simulink library "ammclib_bam_S32K3xx"  (R2016a)
(part 23 of 50)

      |     delete_block([gcb, '/fltInK_1_D']);
      |     add_block('built-in/Inport', [gcb, '/fltInK_1_D'], 'Position', pos, 'Orientation', orient, 'OutDataTypeStr', 'single');
      | 
      |     pos = get_param([gcb, '/fltPropGain_Q'], 'Position');
      |     orient = get_param([gcb, '/fltPropGain_Q'], 'Orientation');
      |     delete_block([gcb, '/fltPropGain_Q']);
      |     add_block('built-in/Inport', [gcb, '/fltPropGain_Q'], 'Position', pos, 'Orientation', orient, 'OutDataTypeStr', 'single');
      | 
      |     pos = get_param([gcb, '/fltIntegGain_Q'], 'Position');
      |     orient = get_param([gcb, '/fltIntegGain_Q'], 'Orientation');
      |     delete_block([gcb, '/fltIntegGain_Q']);
      |     add_block('built-in/Inport', [gcb, '/fltIntegGain_Q'], 'Position', pos, 'Orientation', orient, 'OutDataTypeStr', 'single');
      | 
      |     pos = get_param([gcb, '/fltIntegPartK_1_Q'], 'Position');
      |     orient = get_param([gcb, '/fltIntegPartK_1_Q'], 'Orientation');
      |     delete_block([gcb, '/fltIntegPartK_1_Q']);
      |     add_block('built-in/Inport', [gcb, '/fltIntegPartK_1_Q'], 'Position', pos, 'Orientation', orient, 'OutDataTypeStr', 'single');
      | 
      |     pos = get_param([gcb, '/fltInK_1_Q'], 'Position');
      |     orient = get_param([gcb, '/fltInK_1_Q'], 'Orientation');
      |     delete_block([gcb, '/fltInK_1_Q']);
      |     add_block('built-in/Inport', [gcb, '/fltInK_1_Q'], 'Position', pos, 'Orientation', orient, 'OutDataTypeStr', 'single');
      | 
      | 
      | 
      |     pos = get_param([gcb '/fltIntegPartK_1_D_Out'], 'Position');
      |     orient = get_param([gcb '/fltIntegPartK_1_D_Out'], 'Orientation');
      |     delete_block([gcb '/fltIntegPartK_1_D_Out']);
      |     add_block('built-in/Outport', [gcb '/fltIntegPartK_1_D_Out'], 'Position', pos, 'Orientation', orient);
      | 
      |     pos = get_param([gcb '/fltInK_1_D_Out'], 'Position');
      |     orient = get_param([gcb '/fltInK_1_D_Out'], 'Orientation');
      |     delete_block([gcb '/fltInK_1_D_Out']);
      |     add_block('built-in/Outport', [gcb '/fltInK_1_D_Out'], 'Position', pos, 'Orientation', orient);
      | 
      |     pos = get_param([gcb '/fltIntegPartK_1_Q_Out'], 'Position');
      |     orient = get_param([gcb '/fltIntegPartK_1_Q_Out'], 'Orientation');
      |     delete_block([gcb '/fltIntegPartK_1_Q_Out']);
      |     add_block('built-in/Outport', [gcb '/fltIntegPartK_1_Q_Out'], 'Position', pos, 'Orientation', orient);
      | 
      |     pos = get_param([gcb '/fltInK_1_Q_Out'], 'Position');
      |     orient = get_param([gcb '/fltInK_1_Q_Out'], 'Orientation');
      |     delete_block([gcb '/fltInK_1_Q_Out']);
      |     add_block('built-in/Outport', [gcb '/fltInK_1_Q_Out'], 'Position', pos, 'Orientation', orient);
      | 
      | 
      |     pmask=Simulink.Mask.get(gcb);
      |     pctrl=pmask.getParameter('SampleTime');
      |     pctrl.set('TypeOptions',{'fltUDcBus/SampleTime','pIDQReq/SampleTime','pIDQFbck/SampleTime','fltControllerPIpAWDOut_preset/SampleTime','fltControllerPIpAWQOut_preset/SampleTime','fltPropGain_D/SampleTime','fltIntegGain_D/SampleTime','fltIntegPartK_1_D/SampleTime','fltInK_1_D/SampleTime','fltPropGain_Q/SampleTime','fltIntegGain_Q/SampleTime','fltIntegPartK_1_Q/SampleTime','fltInK_1_Q/SampleTime'});
      | 
      |     set_param([gcb '/fltUDcBus'], 'Port', '1');
      |     set_param([gcb '/pIDQReq'], 'Port', '2');
      |     set_param([gcb '/pIDQFbck'], 'Port', '3');
      |     set_param([gcb '/fltControllerPIpAWDOut_preset'], 'Port', '4');
      |     set_param([gcb '/fltControllerPIpAWQOut_preset'], 'Port', '5');
      |     set_param([gcb '/fltPropGain_D'], 'Port', '6');
      |     set_param([gcb '/fltIntegGain_D'], 'Port', '7');
      |     set_param([gcb '/fltIntegPartK_1_D'], 'Port', '8');
      |     set_param([gcb '/fltInK_1_D'], 'Port', '9');
      |     set_param([gcb '/fltPropGain_Q'], 'Port', '10');
      |     set_param([gcb '/fltIntegGain_Q'], 'Port', '11');
      |     set_param([gcb '/fltIntegPartK_1_Q'], 'Port', '12');
      |     set_param([gcb '/fltInK_1_Q'], 'Port', '13');
      | 
      |     tmpOutCnt=0;
      |     tmpOutCnt=tmpOutCnt+1;
      |     set_param([gcb '/pUDQReq'], 'Port', num2str(tmpOutCnt));
      |     tmpOutCnt=tmpOutCnt+1;
      |     set_param([gcb '/fltUQLim'], 'Port', num2str(tmpOutCnt));
      |     tmpOutCnt=tmpOutCnt+1;
      |     set_param([gcb '/fltIntegPartK_1_D_Out'], 'Port', num2str(tmpOutCnt));
      |     tmpOutCnt=tmpOutCnt+1;
      |     set_param([gcb '/fltInK_1_D_Out'], 'Port', num2str(tmpOutCnt));
      |     tmpOutCnt=tmpOutCnt+1;
      |     set_param([gcb '/fltIntegPartK_1_Q_Out'], 'Port', num2str(tmpOutCnt));
      |     tmpOutCnt=tmpOutCnt+1;
      |     set_param([gcb '/fltInK_1_Q_Out'], 'Port', num2str(tmpOutCnt));
      | 
      |     set_param(gcb,'MaskEnables',{'on','on','on','off','off','off','off','off','off','off','off','off','off','off'});
      | 
      |     if (posblk(4) - posblk(2)) < 350
      |       height = 350;
      |       set_param(gcb,'Position',[posblk(1), posblk(2), posblk(3), posblk(2)+height])
      |     end
      |   end
      | end
      settings: RTWSystemCode=Inline
      mask Help: web([fileparts(which('ammclib_bam_S32K3xx.slx')) '/../doc/S32K3XXMCLUG.pdf'], '-browser')
      mask TypeOptions showStates: Hide (faster execution) | Show (allows debugging; connect feedback loops manually)
      mask Callback showStates:
      | maskStr=get_param(gcb,'showStates');
      | if strcmp(maskStr,'Hide (faster execution)')
      |   if strcmp(get_param([gcb '/fltPropGain_D'], 'BlockType'), 'Inport')
      |     autoCalcEn=get_param(gcb,'autoCalcEn');
      |     if strcmp(autoCalcEn,'on')
      |       set_param(gcb,'MaskEnables',{'on','on','on','on','on','on','on','on','on','on','on','on','on','off'});
      |     else
      |       set_param(gcb,'MaskEnables',{'on','on','on','off','off','off','off','off','on','on','on','on','on','off'});
      |     end
      |   end
      | else
      |   if strcmp(get_param([gcb '/fltPropGain_D'], 'BlockType'), 'Ground')
      |     set_param(gcb,'MaskEnables',{'on','on','on','off','off','off','off','off','off','off','off','off','off','off'});
      |   end
      | end
      mask TypeOptions resetStatesEnable: Pre-set according to the first set of inputs after reset | Clear to zero
      mask TypeOptions SampleTime: fltUDcBus/SampleTime | pIDQReq/SampleTime | pIDQFbck/SampleTime | fltControllerPIpAWDOut_preset/SampleTime | fltControllerPIpAWQOut_preset/SampleTime
      mask Callback SampleTime:
      | p=Simulink.Mask.get(gcb);
      | hintText=p.getDialogControl('timeHint');
      | SampleTime=Simulink.data.evalinGlobal(bdroot,get_param(gcb,'SampleTime'));
      | SampleTime_1=str2double(get_param(gcb,'SampleTime_1'));
      | if (((SampleTime==-1) && (~contains(hintText.Prompt,'inherited'))) || ...
      |     ((SampleTime~=-1) && contains(hintText.Prompt,'inherited')) || ...
      |     ((SampleTime~=-1) && (SampleTime_1~=SampleTime)) || ...
      |     ((SampleTime_1~=-1) && contains(hintText.Prompt,'yet')))
      |   if ((SampleTime==-1) && (~contains(hintText.Prompt,'inherited')))
      |     set_param(gcb,'SampleTime_1',num2str(NaN));
      |     SampleTime_1=NaN;
      |   end
      |   if (SampleTime~=-1)
      |     set_param(gcb,'SampleTime_1',num2str(SampleTime));
      |     SampleTime_1=SampleTime;
      |   end
      |   autoCalcEn=get_param(gcb,'autoCalcEn');
      |   if strcmp(autoCalcEn,'on')
      |     p=Simulink.Mask.get(gcb);
      |     hintText=p.getDialogControl('timeHint');
      |     if SampleTime==-1
      |       SampleTime=SampleTime_1;
      |       if isnan(SampleTime)
      |         hintText.Prompt='Note: Implementation parameters cannot be calculated yet because the block''s inherited sample time is unknown. Simulink will update the sample time when you run the simulation.';
      |       else
      |         hintText.Prompt='Caution: Implementation parameters depend on inherited sample time. Make sure that the sample time of the block''s inputs corresponds to the sampling period in the target application.';
      |       end
      |     else
      |       hintText.Prompt='Caution: Implementation parameters depend on the sample time. Make sure that the simulation time step corresponds to the sampling period in the target application.';
      |     end
      |     fltPropGain_D_bkup=get_param(gcb,'fltPropGain_D');
      |     fltIntegGain_D_bkup=get_param(gcb,'fltIntegGain_D');
      |     fltPropGain_Q_bkup=get_param(gcb,'fltPropGain_Q');
      |     fltIntegGain_Q_bkup=get_param(gcb,'fltIntegGain_Q');
      |     if0=Simulink.data.evalinGlobal(bdroot,get_param(gcb,'if0'));
      |     iksi=Simulink.data.evalinGlobal(bdroot,get_param(gcb,'iksi'));
      |     Ld=Simulink.data.evalinGlobal(bdroot,get_param(gcb,'Ld'));
      |     Lq=Simulink.data.evalinGlobal(bdroot,get_param(gcb,'Lq'));
      |     Rs=Simulink.data.evalinGlobal(bdroot,get_param(gcb,'Rs'));
      |     if (if0<=0)
      |       warning('Natural frequency f0 must be positive.');
      |     end
      |     if (iksi<=0)
      |       warning('Current loop attenuation must be positive.');
      |     end
      |     if (iksi>1)
      |       warning('Current loop attenuation must not exceed 1.');
      |     end
      |     if (Ld<=0)
      |       warning('Inductance Ld must be positive.');
      |     end
      |     if (Lq<=0)
      |       warning('Inductance Lq must be positive.');
      |     end
      |     if (Rs<0)
      |       warning('Resistance Rs must be non-negative.');
      |     end
      |     w0=6.283185307179586*if0;
      |     pgainD=2.0*iksi*w0*Ld-Rs;
      |     igainD=w0*w0*Ld;
      |     pgainQ=2.0*iksi*w0*Lq-Rs;
      |     igainQ=w0*w0*Lq;
      |     fltPropGain_D=pgainD;
      |     fltIntegGain_D=igainD*SampleTime*0.5;
      |     fltPropGain_Q=pgainQ;
      |     fltIntegGain_Q=igainQ*SampleTime*0.5;
      |     if isnan(fltPropGain_D)
      |       if ~strcmp(fltPropGain_D_bkup,'0')
      |         set_param(gcb,'fltPropGain_D','0');
      |       end
      |     else
      |       tmps=num2str(fltPropGain_D);
      |       if ~strcmp(fltPropGain_D_bkup,tmps)
      |         set_param(gcb,'fltPropGain_D',tmps);
      |       end
      |     end
      |     if isnan(fltIntegGain_D)
      |       if ~strcmp(fltIntegGain_D_bkup,'0')
      |         set_param(gcb,'fltIntegGain_D','0');
      |       end
      |     else
      |       tmps=num2str(fltIntegGain_D);
      |       if ~strcmp(fltIntegGain_D_bkup,tmps)
      |         set_param(gcb,'fltIntegGain_D',tmps);
      |       end
      |     end
      |     if isnan(fltPropGain_Q)
      |       if ~strcmp(fltPropGain_Q_bkup,'0')
      |         set_param(gcb,'fltPropGain_Q','0');
      |       end
      |     else
      |       tmps=num2str(fltPropGain_Q);
      |       if ~strcmp(fltPropGain_Q_bkup,tmps)
      |         set_param(gcb,'fltPropGain_Q',tmps);
      |       end
      |     end
      |     if isnan(fltIntegGain_Q)
      |       if ~strcmp(fltIntegGain_Q_bkup,'0')
      |         set_param(gcb,'fltIntegGain_Q','0');
      |       end
      |     else
      |       tmps=num2str(fltIntegGain_Q);
      |       if ~strcmp(fltIntegGain_Q_bkup,tmps)
      |         set_param(gcb,'fltIntegGain_Q',tmps);
      |       end
      |     end
      |   end
      | end
      mask Callback if0:
      | autoCalcEn=get_param(gcb,'autoCalcEn');
      | if strcmp(autoCalcEn,'on')
      |   SampleTime=Simulink.data.evalinGlobal(bdroot,get_param(gcb,'SampleTime'));
      |   if (SampleTime==-1)
      |     SampleTime=str2double(get_param(gcb,'SampleTime_1'));
      |   end
      |   fltPropGain_D_bkup=get_param(gcb,'fltPropGain_D');
      |   fltIntegGain_D_bkup=get_param(gcb,'fltIntegGain_D');
      |   fltPropGain_Q_bkup=get_param(gcb,'fltPropGain_Q');
      |   fltIntegGain_Q_bkup=get_param(gcb,'fltIntegGain_Q');
      |   if0=Simulink.data.evalinGlobal(bdroot,get_param(gcb,'if0'));
      |   iksi=Simulink.data.evalinGlobal(bdroot,get_param(gcb,'iksi'));
      |   Ld=Simulink.data.evalinGlobal(bdroot,get_param(gcb,'Ld'));
      |   Lq=Simulink.data.evalinGlobal(bdroot,get_param(gcb,'Lq'));
      |   Rs=Simulink.data.evalinGlobal(bdroot,get_param(gcb,'Rs'));
      |   if (if0<=0)
      |     warning('Natural frequency f0 must be positive.');
      |   end
      |   if (iksi<=0)
      |     warning('Current loop attenuation must be positive.');
      |   end
      |   if (iksi>1)
      |     warning('Current loop attenuation must not exceed 1.');
      |   end
      |   if (Ld<=0)
      |     warning('Inductance Ld must be positive.');
      |   end
      |   if (Lq<=0)
      |     warning('Inductance Lq must be positive.');
      |   end
      |   if (Rs<0)
      |     warning('Resistance Rs must be non-negative.');
      |   end
      |   w0=6.283185307179586*if0;
      |   pgainD=2.0*iksi*w0*Ld-Rs;
      |   igainD=w0*w0*Ld;
      |   pgainQ=2.0*iksi*w0*Lq-Rs;
      |   igainQ=w0*w0*Lq;
      |   fltPropGain_D=pgainD;
      |   fltIntegGain_D=igainD*SampleTime*0.5;
      |   fltPropGain_Q=pgainQ;
      |   fltIntegGain_Q=igainQ*SampleTime*0.5;
      |   if isnan(fltPropGain_D)
      |     if ~strcmp(fltPropGain_D_bkup,'0')
      |       set_param(gcb,'fltPropGain_D','0');
      |     end
      |   else
      |     tmps=num2str(fltPropGain_D);
      |     if ~strcmp(fltPropGain_D_bkup,tmps)
      |       set_param(gcb,'fltPropGain_D',tmps);
      |     end
      |   end
      |   if isnan(fltIntegGain_D)
      |     if ~strcmp(fltIntegGain_D_bkup,'0')
      |       set_param(gcb,'fltIntegGain_D','0');
      |     end
      |   else
      |     tmps=num2str(fltIntegGain_D);
      |     if ~strcmp(fltIntegGain_D_bkup,tmps)
      |       set_param(gcb,'fltIntegGain_D',tmps);
      |     end
      |   end
      |   if isnan(fltPropGain_Q)
      |     if ~strcmp(fltPropGain_Q_bkup,'0')
      |       set_param(gcb,'fltPropGain_Q','0');
      |     end
      |   else
      |     tmps=num2str(fltPropGain_Q);
      |     if ~strcmp(fltPropGain_Q_bkup,tmps)
      |       set_param(gcb,'fltPropGain_Q',tmps);
      |     end
      |   end
      |   if isnan(fltIntegGain_Q)
      |     if ~strcmp(fltIntegGain_Q_bkup,'0')
      |       set_param(gcb,'fltIntegGain_Q','0');
      |     end
      |   else
      |     tmps=num2str(fltIntegGain_Q);
      |     if ~strcmp(fltIntegGain_Q_bkup,tmps)
      |       set_param(gcb,'fltIntegGain_Q',tmps);
      |     end
      |   end
      | end
      mask Callback iksi:
      | autoCalcEn=get_param(gcb,'autoCalcEn');
      | if strcmp(autoCalcEn,'on')
      |   SampleTime=Simulink.data.evalinGlobal(bdroot,get_param(gcb,'SampleTime'));
      |   if (SampleTime==-1)
      |     SampleTime=str2double(get_param(gcb,'SampleTime_1'));
      |   end
      |   fltPropGain_D_bkup=get_param(gcb,'fltPropGain_D');
      |   fltIntegGain_D_bkup=get_param(gcb,'fltIntegGain_D');
      |   fltPropGain_Q_bkup=get_param(gcb,'fltPropGain_Q');
      |   fltIntegGain_Q_bkup=get_param(gcb,'fltIntegGain_Q');
      |   if0=Simulink.data.evalinGlobal(bdroot,get_param(gcb,'if0'));
      |   iksi=Simulink.data.evalinGlobal(bdroot,get_param(gcb,'iksi'));
      |   Ld=Simulink.data.evalinGlobal(bdroot,get_param(gcb,'Ld'));
      |   Lq=Simulink.data.evalinGlobal(bdroot,get_param(gcb,'Lq'));
      |   Rs=Simulink.data.evalinGlobal(bdroot,get_param(gcb,'Rs'));
      |   if (if0<=0)
      |     warning('Natural frequency f0 must be positive.');
      |   end
      |   if (iksi<=0)
      |     warning('Current loop attenuation must be positive.');
      |   end
      |   if (iksi>1)
      |     warning('Current loop attenuation must not exceed 1.');
      |   end
      |   if (Ld<=0)
      |     warning('Inductance Ld must be positive.');
      |   end
      |   if (Lq<=0)
      |     warning('Inductance Lq must be positive.');
      |   end
      |   if (Rs<0)
      |     warning('Resistance Rs must be non-negative.');
      |   end
      |   w0=6.283185307179586*if0;
      |   pgainD=2.0*iksi*w0*Ld-Rs;
      |   igainD=w0*w0*Ld;
      |   pgainQ=2.0*iksi*w0*Lq-Rs;
      |   igainQ=w0*w0*Lq;
      |   fltPropGain_D=pgainD;
      |   fltIntegGain_D=igainD*SampleTime*0.5;
      |   fltPropGain_Q=pgainQ;
      |   fltIntegGain_Q=igainQ*SampleTime*0.5;
      |   if isnan(fltPropGain_D)
      |     if ~strcmp(fltPropGain_D_bkup,'0')
      |       set_param(gcb,'fltPropGain_D','0');
      |     end
      |   else
      |     tmps=num2str(fltPropGain_D);
      |     if ~strcmp(fltPropGain_D_bkup,tmps)
      |       set_param(gcb,'fltPropGain_D',tmps);
      |     end
      |   end
      |   if isnan(fltIntegGain_D)
      |     if ~strcmp(fltIntegGain_D_bkup,'0')
      |       set_param(gcb,'fltIntegGain_D','0');
      |     end
      |   else
      |     tmps=num2str(fltIntegGain_D);
      |     if ~strcmp(fltIntegGain_D_bkup,tmps)
      |       set_param(gcb,'fltIntegGain_D',tmps);
      |     end
      |   end
      |   if isnan(fltPropGain_Q)
      |     if ~strcmp(fltPropGain_Q_bkup,'0')
      |       set_param(gcb,'fltPropGain_Q','0');
      |     end
      |   else
      |     tmps=num2str(fltPropGain_Q);
      |     if ~strcmp(fltPropGain_Q_bkup,tmps)
      |       set_param(gcb,'fltPropGain_Q',tmps);
      |     end
      |   end
      |   if isnan(fltIntegGain_Q)
      |     if ~strcmp(fltIntegGain_Q_bkup,'0')
      |       set_param(gcb,'fltIntegGain_Q','0');
      |     end
      |   else
      |     tmps=num2str(fltIntegGain_Q);
      |     if ~strcmp(fltIntegGain_Q_bkup,tmps)
      |       set_param(gcb,'fltIntegGain_Q',tmps);
      |     end
      |   end
      | end
      mask Callback Ld:
      | autoCalcEn=get_param(gcb,'autoCalcEn');
      | if strcmp(autoCalcEn,'on')
      |   SampleTime=Simulink.data.evalinGlobal(bdroot,get_param(gcb,'SampleTime'));
      |   if (SampleTime==-1)
      |     SampleTime=str2double(get_param(gcb,'SampleTime_1'));
      |   end
      |   fltPropGain_D_bkup=get_param(gcb,'fltPropGain_D');
      |   fltIntegGain_D_bkup=get_param(gcb,'fltIntegGain_D');
      |   fltPropGain_Q_bkup=get_param(gcb,'fltPropGain_Q');
      |   fltIntegGain_Q_bkup=get_param(gcb,'fltIntegGain_Q');
      |   if0=Simulink.data.evalinGlobal(bdroot,get_param(gcb,'if0'));
      |   iksi=Simulink.data.evalinGlobal(bdroot,get_param(gcb,'iksi'));
      |   Ld=Simulink.data.evalinGlobal(bdroot,get_param(gcb,'Ld'));
      |   Lq=Simulink.data.evalinGlobal(bdroot,get_param(gcb,'Lq'));
      |   Rs=Simulink.data.evalinGlobal(bdroot,get_param(gcb,'Rs'));
      |   if (if0<=0)
      |     warning('Natural frequency f0 must be positive.');
      |   end
      |   if (iksi<=0)
      |     warning('Current loop attenuation must be positive.');
      |   end
      |   if (iksi>1)
      |     warning('Current loop attenuation must not exceed 1.');
      |   end
      |   if (Ld<=0)
      |     warning('Inductance Ld must be positive.');
      |   end
      |   if (Lq<=0)
      |     warning('Inductance Lq must be positive.');
      |   end
      |   if (Rs<0)
      |     warning('Resistance Rs must be non-negative.');
      |   end
      |   w0=6.283185307179586*if0;
      |   pgainD=2.0*iksi*w0*Ld-Rs;
      |   igainD=w0*w0*Ld;
      |   pgainQ=2.0*iksi*w0*Lq-Rs;
      |   igainQ=w0*w0*Lq;
      |   fltPropGain_D=pgainD;
      |   fltIntegGain_D=igainD*SampleTime*0.5;
      |   fltPropGain_Q=pgainQ;
      |   fltIntegGain_Q=igainQ*SampleTime*0.5;
      |   if isnan(fltPropGain_D)
      |     if ~strcmp(fltPropGain_D_bkup,'0')
      |       set_param(gcb,'fltPropGain_D','0');
      |     end
      |   else
      |     tmps=num2str(fltPropGain_D);
      |     if ~strcmp(fltPropGain_D_bkup,tmps)
      |       set_param(gcb,'fltPropGain_D',tmps);
      |     end
      |   end
      |   if isnan(fltIntegGain_D)
      |     if ~strcmp(fltIntegGain_D_bkup,'0')
      |       set_param(gcb,'fltIntegGain_D','0');
      |     end
      |   else
      |     tmps=num2str(fltIntegGain_D);
      |     if ~strcmp(fltIntegGain_D_bkup,tmps)
      |       set_param(gcb,'fltIntegGain_D',tmps);
      |     end
      |   end
      |   if isnan(fltPropGain_Q)
      |     if ~strcmp(fltPropGain_Q_bkup,'0')
      |       set_param(gcb,'fltPropGain_Q','0');
      |     end
      |   else
      |     tmps=num2str(fltPropGain_Q);
      |     if ~strcmp(fltPropGain_Q_bkup,tmps)
      |       set_param(gcb,'fltPropGain_Q',tmps);
      |     end
      |   end
      |   if isnan(fltIntegGain_Q)
      |     if ~strcmp(fltIntegGain_Q_bkup,'0')
      |       set_param(gcb,'fltIntegGain_Q','0');
      |     end
      |   else
      |     tmps=num2str(fltIntegGain_Q);
      |     if ~strcmp(fltIntegGain_Q_bkup,tmps)
      |       set_param(gcb,'fltIntegGain_Q',tmps);
      |     end
      |   end
      | end
      mask Callback Lq:
      | autoCalcEn=get_param(gcb,'autoCalcEn');
      | if strcmp(autoCalcEn,'on')
      |   SampleTime=Simulink.data.evalinGlobal(bdroot,get_param(gcb,'SampleTime'));
      |   if (SampleTime==-1)
      |     SampleTime=str2double(get_param(gcb,'SampleTime_1'));
      |   end
      |   fltPropGain_D_bkup=get_param(gcb,'fltPropGain_D');
      |   fltIntegGain_D_bkup=get_param(gcb,'fltIntegGain_D');
      |   fltPropGain_Q_bkup=get_param(gcb,'fltPropGain_Q');
      |   fltIntegGain_Q_bkup=get_param(gcb,'fltIntegGain_Q');
      |   if0=Simulink.data.evalinGlobal(bdroot,get_param(gcb,'if0'));
      |   iksi=Simulink.data.evalinGlobal(bdroot,get_param(gcb,'iksi'));
      |   Ld=Simulink.data.evalinGlobal(bdroot,get_param(gcb,'Ld'));
      |   Lq=Simulink.data.evalinGlobal(bdroot,get_param(gcb,'Lq'));
      |   Rs=Simulink.data.evalinGlobal(bdroot,get_param(gcb,'Rs'));
      |   if (if0<=0)
      |     warning('Natural frequency f0 must be positive.');
      |   end
      |   if (iksi<=0)
      |     warning('Current loop attenuation must be positive.');
      |   end
      |   if (iksi>1)
      |     warning('Current loop attenuation must not exceed 1.');
      |   end
      |   if (Ld<=0)
      |     warning('Inductance Ld must be positive.');
      |   end
      |   if (Lq<=0)
      |     warning('Inductance Lq must be positive.');
      |   end
      |   if (Rs<0)
      |     warning('Resistance Rs must be non-negative.');
      |   end
      |   w0=6.283185307179586*if0;
      |   pgainD=2.0*iksi*w0*Ld-Rs;
      |   igainD=w0*w0*Ld;
      |   pgainQ=2.0*iksi*w0*Lq-Rs;
      |   igainQ=w0*w0*Lq;
      |   fltPropGain_D=pgainD;
      |   fltIntegGain_D=igainD*SampleTime*0.5;
      |   fltPropGain_Q=pgainQ;
      |   fltIntegGain_Q=igainQ*SampleTime*0.5;
      |   if isnan(fltPropGain_D)
      |     if ~strcmp(fltPropGain_D_bkup,'0')
      |       set_param(gcb,'fltPropGain_D','0');
      |     end
      |   else
      |     tmps=num2str(fltPropGain_D);
      |     if ~strcmp(fltPropGain_D_bkup,tmps)
      |       set_param(gcb,'fltPropGain_D',tmps);
      |     end
      |   end
      |   if isnan(fltIntegGain_D)
      |     if ~strcmp(fltIntegGain_D_bkup,'0')
      |       set_param(gcb,'fltIntegGain_D','0');
      |     end
      |   else
      |     tmps=num2str(fltIntegGain_D);
      |     if ~strcmp(fltIntegGain_D_bkup,tmps)
      |       set_param(gcb,'fltIntegGain_D',tmps);
      |     end
      |   end
      |   if isnan(fltPropGain_Q)
      |     if ~strcmp(fltPropGain_Q_bkup,'0')
      |       set_param(gcb,'fltPropGain_Q','0');
      |     end
      |   else
      |     tmps=num2str(fltPropGain_Q);
      |     if ~strcmp(fltPropGain_Q_bkup,tmps)
      |       set_param(gcb,'fltPropGain_Q',tmps);
      |     end
      |   end
      |   if isnan(fltIntegGain_Q)
      |     if ~strcmp(fltIntegGain_Q_bkup,'0')
      |       set_param(gcb,'fltIntegGain_Q','0');
      |     end
      |   else
      |     tmps=num2str(fltIntegGain_Q);
      |     if ~strcmp(fltIntegGain_Q_bkup,tmps)
      |       set_param(gcb,'fltIntegGain_Q',tmps);
      |     end
      |   end
      | end
      mask Callback Rs:
      | autoCalcEn=get_param(gcb,'autoCalcEn');
      | if strcmp(autoCalcEn,'on')
      |   SampleTime=Simulink.data.evalinGlobal(bdroot,get_param(gcb,'SampleTime'));
      |   if (SampleTime==-1)
      |     SampleTime=str2double(get_param(gcb,'SampleTime_1'));
      |   end
      |   fltPropGain_D_bkup=get_param(gcb,'fltPropGain_D');
      |   fltIntegGain_D_bkup=get_param(gcb,'fltIntegGain_D');
      |   fltPropGain_Q_bkup=get_param(gcb,'fltPropGain_Q');
      |   fltIntegGain_Q_bkup=get_param(gcb,'fltIntegGain_Q');
      |   if0=Simulink.data.evalinGlobal(bdroot,get_param(gcb,'if0'));
      |   iksi=Simulink.data.evalinGlobal(bdroot,get_param(gcb,'iksi'));
      |   Ld=Simulink.data.evalinGlobal(bdroot,get_param(gcb,'Ld'));
      |   Lq=Simulink.data.evalinGlobal(bdroot,get_param(gcb,'Lq'));
      |   Rs=Simulink.data.evalinGlobal(bdroot,get_param(gcb,'Rs'));
      |   if (if0<=0)
      |     warning('Natural frequency f0 must be positive.');
      |   end
      |   if (iksi<=0)
      |     warning('Current loop attenuation must be positive.');
      |   end
      |   if (iksi>1)
      |     warning('Current loop attenuation must not exceed 1.');
      |   end
      |   if (Ld<=0)
      |     warning('Inductance Ld must be positive.');
      |   end
      |   if (Lq<=0)
      |     warning('Inductance Lq must be positive.');
      |   end
      |   if (Rs<0)
      |     warning('Resistance Rs must be non-negative.');
      |   end
      |   w0=6.283185307179586*if0;
      |   pgainD=2.0*iksi*w0*Ld-Rs;
      |   igainD=w0*w0*Ld;
      |   pgainQ=2.0*iksi*w0*Lq-Rs;
      |   igainQ=w0*w0*Lq;
      |   fltPropGain_D=pgainD;
      |   fltIntegGain_D=igainD*SampleTime*0.5;
      |   fltPropGain_Q=pgainQ;
      |   fltIntegGain_Q=igainQ*SampleTime*0.5;
      |   if isnan(fltPropGain_D)
      |     if ~strcmp(fltPropGain_D_bkup,'0')
      |       set_param(gcb,'fltPropGain_D','0');
      |     end
      |   else
      |     tmps=num2str(fltPropGain_D);
      |     if ~strcmp(fltPropGain_D_bkup,tmps)
      |       set_param(gcb,'fltPropGain_D',tmps);
      |     end
      |   end
      |   if isnan(fltIntegGain_D)
      |     if ~strcmp(fltIntegGain_D_bkup,'0')
      |       set_param(gcb,'fltIntegGain_D','0');
      |     end
      |   else
      |     tmps=num2str(fltIntegGain_D);
      |     if ~strcmp(fltIntegGain_D_bkup,tmps)
      |       set_param(gcb,'fltIntegGain_D',tmps);
      |     end
      |   end
      |   if isnan(fltPropGain_Q)
      |     if ~strcmp(fltPropGain_Q_bkup,'0')
      |       set_param(gcb,'fltPropGain_Q','0');
      |     end
      |   else
      |     tmps=num2str(fltPropGain_Q);
      |     if ~strcmp(fltPropGain_Q_bkup,tmps)
      |       set_param(gcb,'fltPropGain_Q',tmps);
      |     end
      |   end
      |   if isnan(fltIntegGain_Q)
      |     if ~strcmp(fltIntegGain_Q_bkup,'0')
      |       set_param(gcb,'fltIntegGain_Q','0');
      |     end
      |   else
      |     tmps=num2str(fltIntegGain_Q);
      |     if ~strcmp(fltIntegGain_Q_bkup,tmps)
      |       set_param(gcb,'fltIntegGain_Q',tmps);
      |     end
      |   end
      | end
      mask Callback autoCalcEn:
      | maskStr=get_param(gcb,'showStates');
      | if strcmp(maskStr,'Hide (faster execution)')
      |   p=Simulink.Mask.get(gcb);
      |   autoCalcEn=get_param(gcb,'autoCalcEn');
      |   hintText=p.getDialogControl('timeHint');
      |   if strcmp(autoCalcEn,'on')
      |     param=p.getParameter('Rs');
      |     if strcmp(param.Enabled,'off')
      |       SampleTime=Simulink.data.evalinGlobal(bdroot,get_param(gcb,'SampleTime'));
      |       if SampleTime==-1
      |         SampleTime=str2double(get_param(gcb,'SampleTime_1'));
      |         if isnan(SampleTime)
      |           hintText.Prompt=['Note: Implementation parameters cannot be calculated yet because the block''s inherited sample time is unknown. Simulink will update the sample time when you run the simulation.'];
      |         else
      |           hintText.Prompt=['Caution: Implementation parameters depend on inherited sample time. Make sure that the sample time of the block''s inputs corresponds to the sampling period in the target application.'];
      |         end
      |       else
      |         hintText.Prompt='Caution: Implementation parameters depend on the sample time. Make sure that the simulation time step corresponds to the sampling period in the target application.';
      |       end
      |       p=Simulink.Mask.get(gcb);
      |       param=p.getParameter('if0');
      |       param.set('Enabled','on');
      |       param=p.getParameter('iksi');
      |       param.set('Enabled','on');
      |       param=p.getParameter('Ld');
      |       param.set('Enabled','on');
      |       param=p.getParameter('Lq');
      |       param.set('Enabled','on');
      |       param=p.getParameter('Rs');
      |       param.set('Enabled','on');
      |     else
      |       SampleTime=Simulink.data.evalinGlobal(bdroot,get_param(gcb,'SampleTime'));
      |       if SampleTime==-1
      |         SampleTime=str2double(get_param(gcb,'SampleTime_1'));
      |       end
      |     end
      |     fltPropGain_D_bkup=get_param(gcb,'fltPropGain_D');
      |     fltIntegGain_D_bkup=get_param(gcb,'fltIntegGain_D');
      |     fltPropGain_Q_bkup=get_param(gcb,'fltPropGain_Q');
      |     fltIntegGain_Q_bkup=get_param(gcb,'fltIntegGain_Q');
      |     if0=Simulink.data.evalinGlobal(bdroot,get_param(gcb,'if0'));
      |     iksi=Simulink.data.evalinGlobal(bdroot,get_param(gcb,'iksi'));
      |     Ld=Simulink.data.evalinGlobal(bdroot,get_param(gcb,'Ld'));
      |     Lq=Simulink.data.evalinGlobal(bdroot,get_param(gcb,'Lq'));
      |     Rs=Simulink.data.evalinGlobal(bdroot,get_param(gcb,'Rs'));
      |     if (if0<=0)
      |       warning('Natural frequency f0 must be positive.');
      |     end
      |     if (iksi<=0)
      |       warning('Current loop attenuation must be positive.');
      |     end
      |     if (iksi>1)
      |       warning('Current loop attenuation must not exceed 1.');
      |     end
      |     if (Ld<=0)
      |       warning('Inductance Ld must be positive.');
      |     end
      |     if (Lq<=0)
      |       warning('Inductance Lq must be positive.');
      |     end
      |     if (Rs<0)
      |       warning('Resistance Rs must be non-negative.');
      |     end
      |     w0=6.283185307179586*if0;
      |     pgainD=2.0*iksi*w0*Ld-Rs;
      |     igainD=w0*w0*Ld;
      |     pgainQ=2.0*iksi*w0*Lq-Rs;
      |     igainQ=w0*w0*Lq;
      |     fltPropGain_D=pgainD;
      |     fltIntegGain_D=igainD*SampleTime*0.5;
      |     fltPropGain_Q=pgainQ;
      |     fltIntegGain_Q=igainQ*SampleTime*0.5;
      |     if isnan(fltPropGain_D)
      |       if ~strcmp(fltPropGain_D_bkup,'0')
      |         set_param(gcb,'fltPropGain_D','0');
      |       end
      |     else
      |       tmps=num2str(fltPropGain_D);
      |       if ~strcmp(fltPropGain_D_bkup,tmps)
      |         set_param(gcb,'fltPropGain_D',tmps);
      |       end
      |     end
      |     if isnan(fltIntegGain_D)
      |       if ~strcmp(fltIntegGain_D_bkup,'0')
      |         set_param(gcb,'fltIntegGain_D','0');
      |       end
      |     else
      |       tmps=num2str(fltIntegGain_D);
      |       if ~strcmp(fltIntegGain_D_bkup,tmps)
      |         set_param(gcb,'fltIntegGain_D',tmps);
      |       end
      |     end
      |     if isnan(fltPropGain_Q)
      |       if ~strcmp(fltPropGain_Q_bkup,'0')
      |         set_param(gcb,'fltPropGain_Q','0');
      |       end
      |     else
      |       tmps=num2str(fltPropGain_Q);
      |       if ~strcmp(fltPropGain_Q_bkup,tmps)
      |         set_param(gcb,'fltPropGain_Q',tmps);
      |       end
      |     end
      |     if isnan(fltIntegGain_Q)
      |       if ~strcmp(fltIntegGain_Q_bkup,'0')
      |         set_param(gcb,'fltIntegGain_Q','0');
      |       end
      |     else
      |       tmps=num2str(fltIntegGain_Q);
      |       if ~strcmp(fltIntegGain_Q_bkup,tmps)
      |         set_param(gcb,'fltIntegGain_Q',tmps);
      |       end
      |     end
      |   else
      |     param=p.getParameter('Rs');
      |     if strcmp(param.Enabled,'on')
      |       hintText.Prompt='Caution: Implementation parameters are fixed.';
      |       p=Simulink.Mask.get(gcb);
      |       param=p.getParameter('if0');
      |       param.set('Enabled','off');
      |       param=p.getParameter('iksi');
      |       param.set('Enabled','off');
      |       param=p.getParameter('Ld');
      |       param.set('Enabled','off');
      |       param=p.getParameter('Lq');
      |       param.set('Enabled','off');
      |       param=p.getParameter('Rs');
      |       param.set('Enabled','off');
      |     end
      |   end
      | end
      mask DialogControl CompBut Prompt: Recalculate sample times
      mask DialogControl CompBut Tooltip: Simulink updates the sample times of all blocks when the simulation is run. This button will update the sample times now.
      mask DialogControl CompBut Callback:
      | btn=questdlg('This will apply all changes in all open dialog boxes and update the schematic. Do you want to proceed?','Apply all changes','Continue','Cancel','Continue');
      | if strcmp(btn,'Continue')
      |   dlgs=DAStudio.ToolRoot.getOpenDialogs;
      |   for i=1:length(dlgs)
      |     dlgs(i).apply;
      |   end
      |   try
      |     SampleTime_1=str2double(get_param(gcb,'SampleTime_1'));
      |     ts=Simulink.Block.getSampleTimes(gcb);
      |     ts=ts(1).Value(1);
      |     if (SampleTime_1 ~= ts)
      |       SampleTime_1=ts;
      |       set_param(gcb,'SampleTime_1',num2str(ts));
      |       autoCalcEn=get_param(gcb,'autoCalcEn');
      |       if strcmp(autoCalcEn,'on')
      |         SampleTime=Simulink.data.evalinGlobal(bdroot,get_param(gcb,'SampleTime'));
      |         p=Simulink.Mask.get(gcb);
      |         hintText=p.getDialogControl('timeHint');
      |         if SampleTime==-1
      |           SampleTime=SampleTime_1;
      |           hintText.Prompt='Caution: Implementation parameters depend on inherited sample time. Make sure that the sample time of the block''s inputs corresponds to the sampling period in the target application.';
      |         else
      |           hintText.Prompt='Caution: Implementation parameters depend on the sample time. Make sure that the simulation time step corresponds to the sampling period in the target application.';
      |         end
      |         fltPropGain_D_bkup=get_param(gcb,'fltPropGain_D');
      |         fltIntegGain_D_bkup=get_param(gcb,'fltIntegGain_D');
      |         fltPropGain_Q_bkup=get_param(gcb,'fltPropGain_Q');
      |         fltIntegGain_Q_bkup=get_param(gcb,'fltIntegGain_Q');
      |         if0=Simulink.data.evalinGlobal(bdroot,get_param(gcb,'if0'));
      |         iksi=Simulink.data.evalinGlobal(bdroot,get_param(gcb,'iksi'));
      |         Ld=Simulink.data.evalinGlobal(bdroot,get_param(gcb,'Ld'));
      |         Lq=Simulink.data.evalinGlobal(bdroot,get_param(gcb,'Lq'));
      |         Rs=Simulink.data.evalinGlobal(bdroot,get_param(gcb,'Rs'));
      |         if (if0<=0)
      |           warning('Natural frequency f0 must be positive.');
      |         end
      |         if (iksi<=0)
      |           warning('Current loop attenuation must be positive.');
      |         end
      |         if (iksi>1)
      |           warning('Current loop attenuation must not exceed 1.');
      |         end
      |         if (Ld<=0)
      |           warning('Inductance Ld must be positive.');
      |         end
      |         if (Lq<=0)
      |           warning('Inductance Lq must be positive.');
      |         end
      |         if (Rs<0)
      |           warning('Resistance Rs must be non-negative.');
      |         end
      |         w0=6.283185307179586*if0;
      |         pgainD=2.0*iksi*w0*Ld-Rs;
      |         igainD=w0*w0*Ld;
      |         pgainQ=2.0*iksi*w0*Lq-Rs;
      |         igainQ=w0*w0*Lq;
      |         fltPropGain_D=pgainD;
      |         fltIntegGain_D=igainD*SampleTime*0.5;
      |         fltPropGain_Q=pgainQ;
      |         fltIntegGain_Q=igainQ*SampleTime*0.5;
      |         if isnan(fltPropGain_D)
      |           if ~strcmp(fltPropGain_D_bkup,'0')
      |             set_param(gcb,'fltPropGain_D','0');
      |           end
      |         else
      |           tmps=num2str(fltPropGain_D);
      |           if ~strcmp(fltPropGain_D_bkup,tmps)
      |             set_param(gcb,'fltPropGain_D',tmps);
      |           end
      |         end
      |         if isnan(fltIntegGain_D)
      |           if ~strcmp(fltIntegGain_D_bkup,'0')
      |             set_param(gcb,'fltIntegGain_D','0');
      |           end
      |         else
      |           tmps=num2str(fltIntegGain_D);
      |           if ~strcmp(fltIntegGain_D_bkup,tmps)
      |             set_param(gcb,'fltIntegGain_D',tmps);
      |           end
      |         end
      |         if isnan(fltPropGain_Q)
      |           if ~strcmp(fltPropGain_Q_bkup,'0')
      |             set_param(gcb,'fltPropGain_Q','0');
      |           end
      |         else
      |           tmps=num2str(fltPropGain_Q);
      |           if ~strcmp(fltPropGain_Q_bkup,tmps)
      |             set_param(gcb,'fltPropGain_Q',tmps);
      |           end
      |         end
      |         if isnan(fltIntegGain_Q)
      |           if ~strcmp(fltIntegGain_Q_bkup,'0')
      |             set_param(gcb,'fltIntegGain_Q','0');
      |           end
      |         else
      |           tmps=num2str(fltIntegGain_Q);
      |           if ~strcmp(fltIntegGain_Q_bkup,tmps)
      |             set_param(gcb,'fltIntegGain_Q',tmps);
      |           end
      |         end
      |       end
      |     end
      |   catch
      |    warning(['Sample time cannot be calculated for the block ' gcb])
      |   end
      | end
      mask DialogControl timeHint Prompt: Note: Implementation parameters cannot be calculated yet because the block's inherited sample time is unknown. Simulink will update the sample time when you run the simulation.
      mask Display:
      | color('black');
      | pos = get_param(gcb, 'Position');
      | width = pos(3) - pos(1);
      | height = pos(4) - pos(2);
      | tX=width/2;
      | tY=height - 25;
      | color('black');
      | text(tX,tY, 'AMCLIB_CurrentLoopPIp_FLT', 'horizontalAlignment', 'center');
      | if showStates == 2
      |   color('red');
      |   text(tX,tY - 20, ['debugging mode' char(13) char(10) '(limited performance)'], 'horizontalAlignment', 'center');
      | end
  AMCLIB_CurrentLoop_FLT : Subsystem  StartFcn=|  TreatAsAtomicUnit=on  mask(AMCLIB_CurrentLoop_FLT){showStates=Hide (faster execution), resetStatesEnable=Pre-set according to the first set of inputs after reset, SampleTime=-1, intmethod=Trapezoidal, if0=350, iksi=1, Ld=3e-4, Lq=3e-4, Rs=0.33, autoCalcEn=on, fltCC1sc_D=0, fltCC2sc_D=0, fltCC1sc_Q=0, fltCC2sc_Q=0, SampleTime_1=NaN}
      | ts=get_param(gcb,'CompiledSampleTime');
      | if iscell(ts)
      |   ts=ts{1};
      |   if iscell(ts)
      |     ts=ts{1};
      |   end
      | end
      | ts=ts(1);
      | set_param(gcb,'SampleTime_1',num2str(ts));
      | p=Simulink.Mask.get(gcb);
      | hintText=p.getDialogControl('timeHint');
      | SampleTime=Simulink.data.evalinGlobal(bdroot,get_param(gcb,'SampleTime'));
      | p=Simulink.Mask.get(gcb);
      | autoCalcEn=get_param(gcb,'autoCalcEn');
      | if strcmp(autoCalcEn,'on')
      |   if SampleTime==-1
      |     hintText.Prompt='Caution: Implementation parameters depend on inherited sample time. Make sure that the sample time of the block''s inputs corresponds to the sampling period in the target application.';
      |   else
      |     hintText.Prompt='Caution: Implementation parameters depend on the sample time. Make sure that the simulation time step corresponds to the sampling period in the target application.';
      |   end
      |   SampleTime=ts;
      |   fltCC1sc_D_bkup=get_param(gcb,'fltCC1sc_D');
      |   fltCC2sc_D_bkup=get_param(gcb,'fltCC2sc_D');
      |   fltCC1sc_Q_bkup=get_param(gcb,'fltCC1sc_Q');
      |   fltCC2sc_Q_bkup=get_param(gcb,'fltCC2sc_Q');
      |   intmethod=get_param(gcb,'intmethod');
      |   if0=Simulink.data.evalinGlobal(bdroot,get_param(gcb,'if0'));
      |   iksi=Simulink.data.evalinGlobal(bdroot,get_param(gcb,'iksi'));
      |   Ld=Simulink.data.evalinGlobal(bdroot,get_param(gcb,'Ld'));
      |   Lq=Simulink.data.evalinGlobal(bdroot,get_param(gcb,'Lq'));
      |   Rs=Simulink.data.evalinGlobal(bdroot,get_param(gcb,'Rs'));
      |   if (if0<=0)
      |     warning('Natural frequency f0 must be positive.');
      |   end
      |   if (iksi<=0)
      |     warning('Current loop attenuation must be positive.');
      |   end
      |   if (iksi>1)
      |     warning('Current loop attenuation must not exceed 1.');
      |   end
      |   if (Ld<=0)
      |     warning('Inductance Ld must be positive.');
      |   end
      |   if (Lq<=0)
      |     warning('Inductance Lq must be positive.');
      |   end
      |   if (Rs<0)
      |     warning('Resistance Rs must be non-negative.');
      |   end
      |   w0=6.283185307179586*if0;
      |   pgainD=2.0*iksi*w0*Ld-Rs;
      |   igainD=w0*w0*Ld;
      |   pgainQ=2.0*iksi*w0*Lq-Rs;
      |   igainQ=w0*w0*Lq;
      |   if strcmp(intmethod,'Forward Rectangular')
      |     cc1d=pgainD;
      |     cc2d=-pgainD+igainD*SampleTime;
      |     cc1q=pgainQ;
      |     cc2q=-pgainQ+igainQ*SampleTime;
      |   else
      |     if strcmp(intmethod,'Backward Rectangular')
      |       cc1d=pgainD+igainD*SampleTime;
      |       cc2d=-pgainD;
      |       cc1q=pgainQ+igainQ*SampleTime;
      |       cc2q=-pgainQ;
      |     else
      |       cc1d=pgainD+igainD*SampleTime*0.5;
      |       cc2d=-pgainD+igainD*SampleTime*0.5;
      |       cc1q=pgainQ+igainQ*SampleTime*0.5;
      |       cc2q=-pgainQ+igainQ*SampleTime*0.5;
      |     end
      |   end
      |   fltCC1sc_D=cc1d;
      |   fltCC2sc_D=cc2d;
      |   fltCC1sc_Q=cc1q;
      |   fltCC2sc_Q=cc2q;
      |   if isnan(fltCC1sc_D)
      |     if ~strcmp(fltCC1sc_D_bkup,'0')
      |       set_param(gcb,'fltCC1sc_D','0');
      |     end
      |   else
      |     tmps=num2str(fltCC1sc_D);
      |     if ~strcmp(fltCC1sc_D_bkup,tmps)
      |       set_param(gcb,'fltCC1sc_D',tmps);
      |     end
      |   end
      |   if isnan(fltCC2sc_D)
      |     if ~strcmp(fltCC2sc_D_bkup,'0')
      |       set_param(gcb,'fltCC2sc_D','0');
      |     end
      |   else
      |     tmps=num2str(fltCC2sc_D);
      |     if ~strcmp(fltCC2sc_D_bkup,tmps)
      |       set_param(gcb,'fltCC2sc_D',tmps);
      |     end
      |   end
      |   if isnan(fltCC1sc_Q)
      |     if ~strcmp(fltCC1sc_Q_bkup,'0')
      |       set_param(gcb,'fltCC1sc_Q','0');
      |     end
      |   else
      |     tmps=num2str(fltCC1sc_Q);
      |     if ~strcmp(fltCC1sc_Q_bkup,tmps)
      |       set_param(gcb,'fltCC1sc_Q',tmps);
      |     end
      |   end
      |   if isnan(fltCC2sc_Q)
      |     if ~strcmp(fltCC2sc_Q_bkup,'0')
      |       set_param(gcb,'fltCC2sc_Q','0');
      |     end
      |   else
      |     tmps=num2str(fltCC2sc_Q);
      |     if ~strcmp(fltCC2sc_Q_bkup,tmps)
      |       set_param(gcb,'fltCC2sc_Q',tmps);
      |     end
      |   end
      | end
      mask prompts: showStates "Show internal states:"; resetStatesEnable "Internal state after reset:"; SampleTime "Sample time (-1 for inherited):"; intmethod "Integration method:"; if0 "Current loop natural frequency f0 [Hz]:"; iksi "Current loop attenuation ξ:"; Ld "D-axis stator inductance Ld [H]"; Lq "Q-axis stator inductance Lq [H]"; Rs "Winding resistance Rs [ohm]:"; autoCalcEn "Calculate implementation parameters from physical parameters"; fltCC1sc_D "fltCC1sc_D (CC1 coefficient of the D-axis PI controller):"; fltCC2sc_D "fltCC2sc_D (CC2 coefficient of the D-axis PI controller):"; fltCC1sc_Q "fltCC1sc_Q (CC1 coefficient of the Q-axis PI controller):"; fltCC2sc_Q "fltCC2sc_Q (CC2 coefficient of the Q-axis PI controller):"; SampleTime_1 "Discrete sample time:"
      mask help: Current control loop of the PMSM field-oriented control algorithm in single precision floating-point implementation. The current control loop contains two PI controllers in recurrent form. This block supports re-initialization of the internal state during simulation. If the block is reset, the outputs of the PI controllers will be aligned with the inputs fltControllerPIrAWDOut_preset and fltControllerPIrAWQOut_preset. Refer to the AMMCLIB User's Guide for further details.
      mask init:
      | ddName = get_param(bdroot,'DataDictionary');
      | if length(ddName)==0
      |   set_param(bdroot,'DataDictionary','ammclib_types.sldd');
      | else
      |   dd = Simulink.data.dictionary.open(ddName);
      |   data = getSection(dd,'Design Data');
      |   if ~exist(data,'SWLIBS_2Syst_F16')
      |     addDataSource(dd,'ammclib_types.sldd');
      |     saveChanges(dd);
      |   end
      | end
      | 
      | if showStates == 1
      |   % hidden state variables
      |   if strcmp(get_param([gcb '/fltCC1sc_D'], 'BlockType'), 'Inport')
      |     posblk = get_param(gcb, 'Position');
      | 
      |     pos = get_param([gcb, '/fltCC1sc_D'], 'Position');
      |     orient = get_param([gcb, '/fltCC1sc_D'], 'Orientation');
      |     delete_block([gcb, '/fltCC1sc_D']);
      |     add_block('built-in/Ground', [gcb, '/fltCC1sc_D'], 'Position', pos, 'Orientation', orient);
      | 
      |     pos = get_param([gcb, '/fltCC2sc_D'], 'Position');
      |     orient = get_param([gcb, '/fltCC2sc_D'], 'Orientation');
      |     delete_block([gcb, '/fltCC2sc_D']);
      |     add_block('built-in/Ground', [gcb, '/fltCC2sc_D'], 'Position', pos, 'Orientation', orient);
      | 
      |     pos = get_param([gcb, '/fltCC1sc_Q'], 'Position');
      |     orient = get_param([gcb, '/fltCC1sc_Q'], 'Orientation');
      |     delete_block([gcb, '/fltCC1sc_Q']);
      |     add_block('built-in/Ground', [gcb, '/fltCC1sc_Q'], 'Position', pos, 'Orientation', orient);
      | 
      |     pos = get_param([gcb, '/fltCC2sc_Q'], 'Position');
      |     orient = get_param([gcb, '/fltCC2sc_Q'], 'Orientation');
      |     delete_block([gcb, '/fltCC2sc_Q']);
      |     add_block('built-in/Ground', [gcb, '/fltCC2sc_Q'], 'Position', pos, 'Orientation', orient);
      | 
      |     pos = get_param([gcb, '/fltAcc_D'], 'Position');
      |     orient = get_param([gcb, '/fltAcc_D'], 'Orientation');
      |     delete_block([gcb, '/fltAcc_D']);
      |     add_block('built-in/Ground', [gcb, '/fltAcc_D'], 'Position', pos, 'Orientation', orient);
      | 
      |     pos = get_param([gcb, '/fltInErrK1_D'], 'Position');
      |     orient = get_param([gcb, '/fltInErrK1_D'], 'Orientation');
      |     delete_block([gcb, '/fltInErrK1_D']);
      |     add_block('built-in/Ground', [gcb, '/fltInErrK1_D'], 'Position', pos, 'Orientation', orient);
      | 
      |     pos = get_param([gcb, '/fltAcc_Q'], 'Position');
      |     orient = get_param([gcb, '/fltAcc_Q'], 'Orientation');
      |     delete_block([gcb, '/fltAcc_Q']);
      |     add_block('built-in/Ground', [gcb, '/fltAcc_Q'], 'Position', pos, 'Orientation', orient);
      | 
      |     pos = get_param([gcb, '/fltInErrK1_Q'], 'Position');
      |     orient = get_param([gcb, '/fltInErrK1_Q'], 'Orientation');
      |     delete_block([gcb, '/fltInErrK1_Q']);
      |     add_block('built-in/Ground', [gcb, '/fltInErrK1_Q'], 'Position', pos, 'Orientation', orient);
      | 
      | 
      |     pmask=Simulink.Mask.get(gcb);
      |     pctrl=pmask.getParameter('SampleTime');
      |     pctrl.set('TypeOptions',{'fltUDcBus/SampleTime','pIDQReq/SampleTime','pIDQFbck/SampleTime','fltControllerPIrAWDOut_preset/SampleTime','fltControllerPIrAWQOut_preset/SampleTime'});
      | 
      |     pos = get_param([gcb '/fltAcc_D_Out'], 'Position');
      |     orient = get_param([gcb '/fltAcc_D_Out'], 'Orientation');
      |     delete_block([gcb '/fltAcc_D_Out']);
      |     add_block('built-in/Terminator', [gcb '/fltAcc_D_Out'], 'Position', pos, 'Orientation', orient);
      | 
      |     pos = get_param([gcb '/fltInErrK1_D_Out'], 'Position');
      |     orient = get_param([gcb '/fltInErrK1_D_Out'], 'Orientation');
      |     delete_block([gcb '/fltInErrK1_D_Out']);
      |     add_block('built-in/Terminator', [gcb '/fltInErrK1_D_Out'], 'Position', pos, 'Orientation', orient);
      | 
      |     pos = get_param([gcb '/fltAcc_Q_Out'], 'Position');
      |     orient = get_param([gcb '/fltAcc_Q_Out'], 'Orientation');
      |     delete_block([gcb '/fltAcc_Q_Out']);
      |     add_block('built-in/Terminator', [gcb '/fltAcc_Q_Out'], 'Position', pos, 'Orientation', orient);
      | 
      |     pos = get_param([gcb '/fltInErrK1_Q_Out'], 'Position');
      |     orient = get_param([gcb '/fltInErrK1_Q_Out'], 'Orientation');
      |     delete_block([gcb '/fltInErrK1_Q_Out']);
      |     add_block('built-in/Terminator', [gcb '/fltInErrK1_Q_Out'], 'Position', pos, 'Orientation', orient);
      | 
      |     set_param([gcb '/fltUDcBus'], 'Port', '1');
      |     set_param([gcb '/pIDQReq'], 'Port', '2');
      |     set_param([gcb '/pIDQFbck'], 'Port', '3');
      |     set_param([gcb '/fltControllerPIrAWDOut_preset'], 'Port', '4');
      |     set_param([gcb '/fltControllerPIrAWQOut_preset'], 'Port', '5');
      | 
      |     tmpOutCnt=0;
      |     tmpOutCnt=tmpOutCnt+1;
      |     set_param([gcb '/pUDQReq'], 'Port', num2str(tmpOutCnt));
      |     tmpOutCnt=tmpOutCnt+1;
      |     set_param([gcb '/fltUQLim'], 'Port', num2str(tmpOutCnt));
      | 
      |     autoCalcEn=get_param(gcb,'autoCalcEn');
      |     if strcmp(autoCalcEn,'on')
      |       set_param(gcb,'MaskEnables',{'on','on','on','on','on','on','on','on','on','on','on','on','on','on','off'});
      |     else
      |       set_param(gcb,'MaskEnables',{'on','on','on','off','off','off','off','off','off','on','on','on','on','on','off'});
      |     end
      | 
      |     if (posblk(4) - posblk(2)) > 150
      |       height = 150;
      |       set_param(gcb,'Position',[posblk(1), posblk(2), posblk(3), posblk(2)+height])
      |     end
      |   end
      | else
      |   % shown state variables
      |   if strcmp(get_param([gcb '/fltCC1sc_D'], 'BlockType'), 'Ground')
      |     posblk = get_param(gcb, 'Position');
      | 
      |     pos = get_param([gcb, '/fltCC1sc_D'], 'Position');
      |     orient = get_param([gcb, '/fltCC1sc_D'], 'Orientation');
      |     delete_block([gcb, '/fltCC1sc_D']);
      |     add_block('built-in/Inport', [gcb, '/fltCC1sc_D'], 'Position', pos, 'Orientation', orient, 'OutDataTypeStr', 'single');
      | 
      |     pos = get_param([gcb, '/fltCC2sc_D'], 'Position');
      |     orient = get_param([gcb, '/fltCC2sc_D'], 'Orientation');
      |     delete_block([gcb, '/fltCC2sc_D']);
      |     add_block('built-in/Inport', [gcb, '/fltCC2sc_D'], 'Position', pos, 'Orientation', orient, 'OutDataTypeStr', 'single');
      | 
      |     pos = get_param([gcb, '/fltCC1sc_Q'], 'Position');
      |     orient = get_param([gcb, '/fltCC1sc_Q'], 'Orientation');
      |     delete_block([gcb, '/fltCC1sc_Q']);
      |     add_block('built-in/Inport', [gcb, '/fltCC1sc_Q'], 'Position', pos, 'Orientation', orient, 'OutDataTypeStr', 'single');
      | 
      |     pos = get_param([gcb, '/fltCC2sc_Q'], 'Position');
      |     orient = get_param([gcb, '/fltCC2sc_Q'], 'Orientation');
      |     delete_block([gcb, '/fltCC2sc_Q']);
      |     add_block('built-in/Inport', [gcb, '/fltCC2sc_Q'], 'Position', pos, 'Orientation', orient, 'OutDataTypeStr', 'single');
      | 
      |     pos = get_param([gcb, '/fltAcc_D'], 'Position');
      |     orient = get_param([gcb, '/fltAcc_D'], 'Orientation');
      |     delete_block([gcb, '/fltAcc_D']);
      |     add_block('built-in/Inport', [gcb, '/fltAcc_D'], 'Position', pos, 'Orientation', orient, 'OutDataTypeStr', 'single');
      | 
      |     pos = get_param([gcb, '/fltInErrK1_D'], 'Position');
      |     orient = get_param([gcb, '/fltInErrK1_D'], 'Orientation');
      |     delete_block([gcb, '/fltInErrK1_D']);
      |     add_block('built-in/Inport', [gcb, '/fltInErrK1_D'], 'Position', pos, 'Orientation', orient, 'OutDataTypeStr', 'single');
      | 
      |     pos = get_param([gcb, '/fltAcc_Q'], 'Position');
      |     orient = get_param([gcb, '/fltAcc_Q'], 'Orientation');
      |     delete_block([gcb, '/fltAcc_Q']);
      |     add_block('built-in/Inport', [gcb, '/fltAcc_Q'], 'Position', pos, 'Orientation', orient, 'OutDataTypeStr', 'single');
      | 
      |     pos = get_param([gcb, '/fltInErrK1_Q'], 'Position');
      |     orient = get_param([gcb, '/fltInErrK1_Q'], 'Orientation');
      |     delete_block([gcb, '/fltInErrK1_Q']);
      |     add_block('built-in/Inport', [gcb, '/fltInErrK1_Q'], 'Position', pos, 'Orientation', orient, 'OutDataTypeStr', 'single');
      | 
      | 
      | 
      |     pos = get_param([gcb '/fltAcc_D_Out'], 'Position');
      |     orient = get_param([gcb '/fltAcc_D_Out'], 'Orientation');
      |     delete_block([gcb '/fltAcc_D_Out']);
      |     add_block('built-in/Outport', [gcb '/fltAcc_D_Out'], 'Position', pos, 'Orientation', orient);
      | 
      |     pos = get_param([gcb '/fltInErrK1_D_Out'], 'Position');
      |     orient = get_param([gcb '/fltInErrK1_D_Out'], 'Orientation');
      |     delete_block([gcb '/fltInErrK1_D_Out']);
      |     add_block('built-in/Outport', [gcb '/fltInErrK1_D_Out'], 'Position', pos, 'Orientation', orient);
      | 
      |     pos = get_param([gcb '/fltAcc_Q_Out'], 'Position');
      |     orient = get_param([gcb '/fltAcc_Q_Out'], 'Orientation');
      |     delete_block([gcb '/fltAcc_Q_Out']);
      |     add_block('built-in/Outport', [gcb '/fltAcc_Q_Out'], 'Position', pos, 'Orientation', orient);
      | 
      |     pos = get_param([gcb '/fltInErrK1_Q_Out'], 'Position');
      |     orient = get_param([gcb '/fltInErrK1_Q_Out'], 'Orientation');
      |     delete_block([gcb '/fltInErrK1_Q_Out']);
      |     add_block('built-in/Outport', [gcb '/fltInErrK1_Q_Out'], 'Position', pos, 'Orientation', orient);
      | 
      | 
      |     pmask=Simulink.Mask.get(gcb);
      |     pctrl=pmask.getParameter('SampleTime');
      |     pctrl.set('TypeOptions',{'fltUDcBus/SampleTime','pIDQReq/SampleTime','pIDQFbck/SampleTime','fltControllerPIrAWDOut_preset/SampleTime','fltControllerPIrAWQOut_preset/SampleTime','fltCC1sc_D/SampleTime','fltCC2sc_D/SampleTime','fltCC1sc_Q/SampleTime','fltCC2sc_Q/SampleTime','fltAcc_D/SampleTime','fltInErrK1_D/SampleTime','fltAcc_Q/SampleTime','fltInErrK1_Q/SampleTime'});
      | 
      |     set_param([gcb '/fltUDcBus'], 'Port', '1');
      |     set_param([gcb '/pIDQReq'], 'Port', '2');
      |     set_param([gcb '/pIDQFbck'], 'Port', '3');
      |     set_param([gcb '/fltControllerPIrAWDOut_preset'], 'Port', '4');
      |     set_param([gcb '/fltControllerPIrAWQOut_preset'], 'Port', '5');
      |     set_param([gcb '/fltCC1sc_D'], 'Port', '6');
      |     set_param([gcb '/fltCC2sc_D'], 'Port', '7');
      |     set_param([gcb '/fltCC1sc_Q'], 'Port', '8');
      |     set_param([gcb '/fltCC2sc_Q'], 'Port', '9');
      |     set_param([gcb '/fltAcc_D'], 'Port', '10');
      |     set_param([gcb '/fltInErrK1_D'], 'Port', '11');
      |     set_param([gcb '/fltAcc_Q'], 'Port', '12');
      |     set_param([gcb '/fltInErrK1_Q'], 'Port', '13');
      | 
      |     tmpOutCnt=0;
      |     tmpOutCnt=tmpOutCnt+1;
      |     set_param([gcb '/pUDQReq'], 'Port', num2str(tmpOutCnt));
      |     tmpOutCnt=tmpOutCnt+1;
      |     set_param([gcb '/fltUQLim'], 'Port', num2str(tmpOutCnt));
      |     tmpOutCnt=tmpOutCnt+1;
      |     set_param([gcb '/fltAcc_D_Out'], 'Port', num2str(tmpOutCnt));
      |     tmpOutCnt=tmpOutCnt+1;
      |     set_param([gcb '/fltInErrK1_D_Out'], 'Port', num2str(tmpOutCnt));
      |     tmpOutCnt=tmpOutCnt+1;
      |     set_param([gcb '/fltAcc_Q_Out'], 'Port', num2str(tmpOutCnt));
      |     tmpOutCnt=tmpOutCnt+1;
      |     set_param([gcb '/fltInErrK1_Q_Out'], 'Port', num2str(tmpOutCnt));
      | 
      |     set_param(gcb,'MaskEnables',{'on','on','on','off','off','off','off','off','off','off','off','off','off','off','off'});
      | 
      |     if (posblk(4) - posblk(2)) < 350
      |       height = 350;
      |       set_param(gcb,'Position',[posblk(1), posblk(2), posblk(3), posblk(2)+height])
      |     end
      |   end
      | end
      settings: RTWSystemCode=Inline
      mask Help: web([fileparts(which('ammclib_bam_S32K3xx.slx')) '/../doc/S32K3XXMCLUG.pdf'], '-browser')
      mask TypeOptions showStates: Hide (faster execution) | Show (allows debugging; connect feedback loops manually)
      mask Callback showStates:
      | maskStr=get_param(gcb,'showStates');
      | if strcmp(maskStr,'Hide (faster execution)')
      |   if strcmp(get_param([gcb '/fltCC1sc_D'], 'BlockType'), 'Inport')
      |     autoCalcEn=get_param(gcb,'autoCalcEn');
      |     if strcmp(autoCalcEn,'on')
      |       set_param(gcb,'MaskEnables',{'on','on','on','on','on','on','on','on','on','on','on','on','on','on','off'});
      |     else
      |       set_param(gcb,'MaskEnables',{'on','on','on','off','off','off','off','off','off','on','on','on','on','on','off'});
      |     end
      |   end
      | else
      |   if strcmp(get_param([gcb '/fltCC1sc_D'], 'BlockType'), 'Ground')
      |     set_param(gcb,'MaskEnables',{'on','on','on','off','off','off','off','off','off','off','off','off','off','off','off'});
      |   end
      | end
      mask TypeOptions resetStatesEnable: Pre-set according to the first set of inputs after reset | Clear to zero
      mask TypeOptions SampleTime: fltUDcBus/SampleTime | pIDQReq/SampleTime | pIDQFbck/SampleTime | fltControllerPIrAWDOut_preset/SampleTime | fltControllerPIrAWQOut_preset/SampleTime
      mask Callback SampleTime:
      | p=Simulink.Mask.get(gcb);
      | hintText=p.getDialogControl('timeHint');
      | SampleTime=Simulink.data.evalinGlobal(bdroot,get_param(gcb,'SampleTime'));
      | SampleTime_1=str2double(get_param(gcb,'SampleTime_1'));
      | if (((SampleTime==-1) && (~contains(hintText.Prompt,'inherited'))) || ...
      |     ((SampleTime~=-1) && contains(hintText.Prompt,'inherited')) || ...
      |     ((SampleTime~=-1) && (SampleTime_1~=SampleTime)) || ...
      |     ((SampleTime_1~=-1) && contains(hintText.Prompt,'yet')))
      |   if ((SampleTime==-1) && (~contains(hintText.Prompt,'inherited')))
      |     set_param(gcb,'SampleTime_1',num2str(NaN));
      |     SampleTime_1=NaN;
      |   end
      |   if (SampleTime~=-1)
      |     set_param(gcb,'SampleTime_1',num2str(SampleTime));
      |     SampleTime_1=SampleTime;
      |   end
      |   autoCalcEn=get_param(gcb,'autoCalcEn');
      |   if strcmp(autoCalcEn,'on')
      |     p=Simulink.Mask.get(gcb);
      |     hintText=p.getDialogControl('timeHint');
      |     if SampleTime==-1
      |       SampleTime=SampleTime_1;
      |       if isnan(SampleTime)
      |         hintText.Prompt='Note: Implementation parameters cannot be calculated yet because the block''s inherited sample time is unknown. Simulink will update the sample time when you run the simulation.';
      |       else
      |         hintText.Prompt='Caution: Implementation parameters depend on inherited sample time. Make sure that the sample time of the block''s inputs corresponds to the sampling period in the target application.';
      |       end
      |     else
      |       hintText.Prompt='Caution: Implementation parameters depend on the sample time. Make sure that the simulation time step corresponds to the sampling period in the target application.';
      |     end
      |     fltCC1sc_D_bkup=get_param(gcb,'fltCC1sc_D');
      |     fltCC2sc_D_bkup=get_param(gcb,'fltCC2sc_D');
      |     fltCC1sc_Q_bkup=get_param(gcb,'fltCC1sc_Q');
      |     fltCC2sc_Q_bkup=get_param(gcb,'fltCC2sc_Q');
      |     intmethod=get_param(gcb,'intmethod');
      |     if0=Simulink.data.evalinGlobal(bdroot,get_param(gcb,'if0'));
      |     iksi=Simulink.data.evalinGlobal(bdroot,get_param(gcb,'iksi'));
      |     Ld=Simulink.data.evalinGlobal(bdroot,get_param(gcb,'Ld'));
      |     Lq=Simulink.data.evalinGlobal(bdroot,get_param(gcb,'Lq'));
      |     Rs=Simulink.data.evalinGlobal(bdroot,get_param(gcb,'Rs'));
      |     if (if0<=0)
      |       warning('Natural frequency f0 must be positive.');
      |     end
      |     if (iksi<=0)
      |       warning('Current loop attenuation must be positive.');
      |     end
      |     if (iksi>1)
      |       warning('Current loop attenuation must not exceed 1.');
      |     end
      |     if (Ld<=0)
      |       warning('Inductance Ld must be positive.');
      |     end
      |     if (Lq<=0)
      |       warning('Inductance Lq must be positive.');
      |     end
      |     if (Rs<0)
      |       warning('Resistance Rs must be non-negative.');
      |     end
      |     w0=6.283185307179586*if0;
      |     pgainD=2.0*iksi*w0*Ld-Rs;
      |     igainD=w0*w0*Ld;
      |     pgainQ=2.0*iksi*w0*Lq-Rs;
      |     igainQ=w0*w0*Lq;
      |     if strcmp(intmethod,'Forward Rectangular')
      |       cc1d=pgainD;
      |       cc2d=-pgainD+igainD*SampleTime;
      |       cc1q=pgainQ;
      |       cc2q=-pgainQ+igainQ*SampleTime;
      |     else
      |       if strcmp(intmethod,'Backward Rectangular')
      |         cc1d=pgainD+igainD*SampleTime;
      |         cc2d=-pgainD;
      |         cc1q=pgainQ+igainQ*SampleTime;
      |         cc2q=-pgainQ;
      |       else
      |         cc1d=pgainD+igainD*SampleTime*0.5;
      |         cc2d=-pgainD+igainD*SampleTime*0.5;
      |         cc1q=pgainQ+igainQ*SampleTime*0.5;
      |         cc2q=-pgainQ+igainQ*SampleTime*0.5;
      |       end
      |     end
      |     fltCC1sc_D=cc1d;
      |     fltCC2sc_D=cc2d;
      |     fltCC1sc_Q=cc1q;
      |     fltCC2sc_Q=cc2q;
      |     if isnan(fltCC1sc_D)
      |       if ~strcmp(fltCC1sc_D_bkup,'0')
      |         set_param(gcb,'fltCC1sc_D','0');
      |       end
      |     else
      |       tmps=num2str(fltCC1sc_D);
      |       if ~strcmp(fltCC1sc_D_bkup,tmps)
      |         set_param(gcb,'fltCC1sc_D',tmps);
      |       end
      |     end
      |     if isnan(fltCC2sc_D)
      |       if ~strcmp(fltCC2sc_D_bkup,'0')
      |         set_param(gcb,'fltCC2sc_D','0');
      |       end
      |     else
      |       tmps=num2str(fltCC2sc_D);
      |       if ~strcmp(fltCC2sc_D_bkup,tmps)
      |         set_param(gcb,'fltCC2sc_D',tmps);
      |       end
      |     end
      |     if isnan(fltCC1sc_Q)
      |       if ~strcmp(fltCC1sc_Q_bkup,'0')
      |         set_param(gcb,'fltCC1sc_Q','0');
      |       end
      |     else
      |       tmps=num2str(fltCC1sc_Q);
      |       if ~strcmp(fltCC1sc_Q_bkup,tmps)
      |         set_param(gcb,'fltCC1sc_Q',tmps);
      |       end
      |     end
      |     if isnan(fltCC2sc_Q)
      |       if ~strcmp(fltCC2sc_Q_bkup,'0')
      |         set_param(gcb,'fltCC2sc_Q','0');
      |       end
      |     else
      |       tmps=num2str(fltCC2sc_Q);
      |       if ~strcmp(fltCC2sc_Q_bkup,tmps)
      |         set_param(gcb,'fltCC2sc_Q',tmps);
      |       end
      |     end
      |   end
      | end
      mask TypeOptions intmethod: Forward Rectangular | Backward Rectangular | Trapezoidal
      mask Callback intmethod:
      | autoCalcEn=get_param(gcb,'autoCalcEn');
      | if strcmp(autoCalcEn,'on')
      |   SampleTime=Simulink.data.evalinGlobal(bdroot,get_param(gcb,'SampleTime'));
      |   if (SampleTime==-1)
      |     SampleTime=str2double(get_param(gcb,'SampleTime_1'));
      |   end
      |   fltCC1sc_D_bkup=get_param(gcb,'fltCC1sc_D');
      |   fltCC2sc_D_bkup=get_param(gcb,'fltCC2sc_D');
      |   fltCC1sc_Q_bkup=get_param(gcb,'fltCC1sc_Q');
      |   fltCC2sc_Q_bkup=get_param(gcb,'fltCC2sc_Q');
      |   intmethod=get_param(gcb,'intmethod');
      |   if0=Simulink.data.evalinGlobal(bdroot,get_param(gcb,'if0'));
      |   iksi=Simulink.data.evalinGlobal(bdroot,get_param(gcb,'iksi'));
      |   Ld=Simulink.data.evalinGlobal(bdroot,get_param(gcb,'Ld'));
      |   Lq=Simulink.data.evalinGlobal(bdroot,get_param(gcb,'Lq'));
      |   Rs=Simulink.data.evalinGlobal(bdroot,get_param(gcb,'Rs'));
      |   if (if0<=0)
      |     warning('Natural frequency f0 must be positive.');
      |   end
      |   if (iksi<=0)
      |     warning('Current loop attenuation must be positive.');
      |   end
      |   if (iksi>1)
      |     warning('Current loop attenuation must not exceed 1.');
      |   end
      |   if (Ld<=0)
      |     warning('Inductance Ld must be positive.');
      |   end
      |   if (Lq<=0)
      |     warning('Inductance Lq must be positive.');
      |   end
      |   if (Rs<0)
      |     warning('Resistance Rs must be non-negative.');
      |   end
      |   w0=6.283185307179586*if0;
      |   pgainD=2.0*iksi*w0*Ld-Rs;
      |   igainD=w0*w0*Ld;
      |   pgainQ=2.0*iksi*w0*Lq-Rs;
      |   igainQ=w0*w0*Lq;
      |   if strcmp(intmethod,'Forward Rectangular')
      |     cc1d=pgainD;
      |     cc2d=-pgainD+igainD*SampleTime;
      |     cc1q=pgainQ;
      |     cc2q=-pgainQ+igainQ*SampleTime;
      |   else
      |     if strcmp(intmethod,'Backward Rectangular')
      |       cc1d=pgainD+igainD*SampleTime;
      |       cc2d=-pgainD;
      |       cc1q=pgainQ+igainQ*SampleTime;
      |       cc2q=-pgainQ;
      |     else
      |       cc1d=pgainD+igainD*SampleTime*0.5;
      |       cc2d=-pgainD+igainD*SampleTime*0.5;
      |       cc1q=pgainQ+igainQ*SampleTime*0.5;
      |       cc2q=-pgainQ+igainQ*SampleTime*0.5;
      |     end
      |   end
      |   fltCC1sc_D=cc1d;
      |   fltCC2sc_D=cc2d;
      |   fltCC1sc_Q=cc1q;
      |   fltCC2sc_Q=cc2q;
      |   if isnan(fltCC1sc_D)
      |     if ~strcmp(fltCC1sc_D_bkup,'0')
      |       set_param(gcb,'fltCC1sc_D','0');
      |     end
      |   else
      |     tmps=num2str(fltCC1sc_D);
      |     if ~strcmp(fltCC1sc_D_bkup,tmps)
      |       set_param(gcb,'fltCC1sc_D',tmps);
      |     end
      |   end
      |   if isnan(fltCC2sc_D)
      |     if ~strcmp(fltCC2sc_D_bkup,'0')
      |       set_param(gcb,'fltCC2sc_D','0');
      |     end
      |   else
      |     tmps=num2str(fltCC2sc_D);
      |     if ~strcmp(fltCC2sc_D_bkup,tmps)
      |       set_param(gcb,'fltCC2sc_D',tmps);
      |     end
      |   end
      |   if isnan(fltCC1sc_Q)
      |     if ~strcmp(fltCC1sc_Q_bkup,'0')
      |       set_param(gcb,'fltCC1sc_Q','0');
      |     end
      |   else
      |     tmps=num2str(fltCC1sc_Q);
      |     if ~strcmp(fltCC1sc_Q_bkup,tmps)
      |       set_param(gcb,'fltCC1sc_Q',tmps);
      |     end
      |   end
      |   if isnan(fltCC2sc_Q)
      |     if ~strcmp(fltCC2sc_Q_bkup,'0')
      |       set_param(gcb,'fltCC2sc_Q','0');
      |     end
      |   else
      |     tmps=num2str(fltCC2sc_Q);
      |     if ~strcmp(fltCC2sc_Q_bkup,tmps)
      |       set_param(gcb,'fltCC2sc_Q',tmps);
      |     end
      |   end
      | end
      mask Callback if0:
      | autoCalcEn=get_param(gcb,'autoCalcEn');
      | if strcmp(autoCalcEn,'on')
      |   SampleTime=Simulink.data.evalinGlobal(bdroot,get_param(gcb,'SampleTime'));
      |   if (SampleTime==-1)
      |     SampleTime=str2double(get_param(gcb,'SampleTime_1'));
      |   end
      |   fltCC1sc_D_bkup=get_param(gcb,'fltCC1sc_D');
      |   fltCC2sc_D_bkup=get_param(gcb,'fltCC2sc_D');
      |   fltCC1sc_Q_bkup=get_param(gcb,'fltCC1sc_Q');
      |   fltCC2sc_Q_bkup=get_param(gcb,'fltCC2sc_Q');
      |   intmethod=get_param(gcb,'intmethod');
      |   if0=Simulink.data.evalinGlobal(bdroot,get_param(gcb,'if0'));
      |   iksi=Simulink.data.evalinGlobal(bdroot,get_param(gcb,'iksi'));
      |   Ld=Simulink.data.evalinGlobal(bdroot,get_param(gcb,'Ld'));
      |   Lq=Simulink.data.evalinGlobal(bdroot,get_param(gcb,'Lq'));
      |   Rs=Simulink.data.evalinGlobal(bdroot,get_param(gcb,'Rs'));
      |   if (if0<=0)
      |     warning('Natural frequency f0 must be positive.');
      |   end
      |   if (iksi<=0)
      |     warning('Current loop attenuation must be positive.');
      |   end
      |   if (iksi>1)
      |     warning('Current loop attenuation must not exceed 1.');
      |   end
      |   if (Ld<=0)
      |     warning('Inductance Ld must be positive.');
      |   end
      |   if (Lq<=0)
      |     warning('Inductance Lq must be positive.');
      |   end
      |   if (Rs<0)
      |     warning('Resistance Rs must be non-negative.');
      |   end
      |   w0=6.283185307179586*if0;
      |   pgainD=2.0*iksi*w0*Ld-Rs;
      |   igainD=w0*w0*Ld;
      |   pgainQ=2.0*iksi*w0*Lq-Rs;
      |   igainQ=w0*w0*Lq;
      |   if strcmp(intmethod,'Forward Rectangular')
      |     cc1d=pgainD;
      |     cc2d=-pgainD+igainD*SampleTime;
      |     cc1q=pgainQ;
      |     cc2q=-pgainQ+igainQ*SampleTime;
      |   else
      |     if strcmp(intmethod,'Backward Rectangular')
      |       cc1d=pgainD+igainD*SampleTime;
      |       cc2d=-pgainD;
      |       cc1q=pgainQ+igainQ*SampleTime;
      |       cc2q=-pgainQ;
      |     else
      |       cc1d=pgainD+igainD*SampleTime*0.5;
      |       cc2d=-pgainD+igainD*SampleTime*0.5;
      |       cc1q=pgainQ+igainQ*SampleTime*0.5;
      |       cc2q=-pgainQ+igainQ*SampleTime*0.5;
      |     end
      |   end
      |   fltCC1sc_D=cc1d;
      |   fltCC2sc_D=cc2d;
      |   fltCC1sc_Q=cc1q;
      |   fltCC2sc_Q=cc2q;
      |   if isnan(fltCC1sc_D)
      |     if ~strcmp(fltCC1sc_D_bkup,'0')
      |       set_param(gcb,'fltCC1sc_D','0');
      |     end
      |   else
      |     tmps=num2str(fltCC1sc_D);
      |     if ~strcmp(fltCC1sc_D_bkup,tmps)
      |       set_param(gcb,'fltCC1sc_D',tmps);
      |     end
      |   end
      |   if isnan(fltCC2sc_D)
      |     if ~strcmp(fltCC2sc_D_bkup,'0')
      |       set_param(gcb,'fltCC2sc_D','0');
      |     end
      |   else
      |     tmps=num2str(fltCC2sc_D);
      |     if ~strcmp(fltCC2sc_D_bkup,tmps)
      |       set_param(gcb,'fltCC2sc_D',tmps);
      |     end
      |   end
      |   if isnan(fltCC1sc_Q)
      |     if ~strcmp(fltCC1sc_Q_bkup,'0')
      |       set_param(gcb,'fltCC1sc_Q','0');
      |     end
      |   else
      |     tmps=num2str(fltCC1sc_Q);
      |     if ~strcmp(fltCC1sc_Q_bkup,tmps)
      |       set_param(gcb,'fltCC1sc_Q',tmps);
      |     end
      |   end
      |   if isnan(fltCC2sc_Q)
      |     if ~strcmp(fltCC2sc_Q_bkup,'0')
      |       set_param(gcb,'fltCC2sc_Q','0');
      |     end
      |   else
      |     tmps=num2str(fltCC2sc_Q);
      |     if ~strcmp(fltCC2sc_Q_bkup,tmps)
      |       set_param(gcb,'fltCC2sc_Q',tmps);
      |     end
      |   end
      | end
      mask Callback iksi:
      | autoCalcEn=get_param(gcb,'autoCalcEn');
      | if strcmp(autoCalcEn,'on')
      |   SampleTime=Simulink.data.evalinGlobal(bdroot,get_param(gcb,'SampleTime'));
      |   if (SampleTime==-1)
      |     SampleTime=str2double(get_param(gcb,'SampleTime_1'));
      |   end
      |   fltCC1sc_D_bkup=get_param(gcb,'fltCC1sc_D');
      |   fltCC2sc_D_bkup=get_param(gcb,'fltCC2sc_D');
      |   fltCC1sc_Q_bkup=get_param(gcb,'fltCC1sc_Q');
      |   fltCC2sc_Q_bkup=get_param(gcb,'fltCC2sc_Q');
      |   intmethod=get_param(gcb,'intmethod');
      |   if0=Simulink.data.evalinGlobal(bdroot,get_param(gcb,'if0'));
      |   iksi=Simulink.data.evalinGlobal(bdroot,get_param(gcb,'iksi'));
      |   Ld=Simulink.data.evalinGlobal(bdroot,get_param(gcb,'Ld'));
      |   Lq=Simulink.data.evalinGlobal(bdroot,get_param(gcb,'Lq'));
      |   Rs=Simulink.data.evalinGlobal(bdroot,get_param(gcb,'Rs'));
      |   if (if0<=0)
      |     warning('Natural frequency f0 must be positive.');
      |   end
      |   if (iksi<=0)
      |     warning('Current loop attenuation must be positive.');
      |   end
      |   if (iksi>1)
      |     warning('Current loop attenuation must not exceed 1.');
      |   end
      |   if (Ld<=0)
      |     warning('Inductance Ld must be positive.');
      |   end
      |   if (Lq<=0)
      |     warning('Inductance Lq must be positive.');
      |   end
      |   if (Rs<0)
      |     warning('Resistance Rs must be non-negative.');
      |   end
      |   w0=6.283185307179586*if0;
      |   pgainD=2.0*iksi*w0*Ld-Rs;
      |   igainD=w0*w0*Ld;
      |   pgainQ=2.0*iksi*w0*Lq-Rs;
      |   igainQ=w0*w0*Lq;
      |   if strcmp(intmethod,'Forward Rectangular')
      |     cc1d=pgainD;
      |     cc2d=-pgainD+igainD*SampleTime;
      |     cc1q=pgainQ;
      |     cc2q=-pgainQ+igainQ*SampleTime;
      |   else
      |     if strcmp(intmethod,'Backward Rectangular')
      |       cc1d=pgainD+igainD*SampleTime;
      |       cc2d=-pgainD;
      |       cc1q=pgainQ+igainQ*SampleTime;
      |       cc2q=-pgainQ;
      |     else
      |       cc1d=pgainD+igainD*SampleTime*0.5;
      |       cc2d=-pgainD+igainD*SampleTime*0.5;
      |       cc1q=pgainQ+igainQ*SampleTime*0.5;
      |       cc2q=-pgainQ+igainQ*SampleTime*0.5;
      |     end
      |   end
      |   fltCC1sc_D=cc1d;
      |   fltCC2sc_D=cc2d;
      |   fltCC1sc_Q=cc1q;
      |   fltCC2sc_Q=cc2q;
      |   if isnan(fltCC1sc_D)
      |     if ~strcmp(fltCC1sc_D_bkup,'0')
      |       set_param(gcb,'fltCC1sc_D','0');
      |     end
      |   else
      |     tmps=num2str(fltCC1sc_D);
      |     if ~strcmp(fltCC1sc_D_bkup,tmps)
      |       set_param(gcb,'fltCC1sc_D',tmps);
      |     end
      |   end
      |   if isnan(fltCC2sc_D)
      |     if ~strcmp(fltCC2sc_D_bkup,'0')
      |       set_param(gcb,'fltCC2sc_D','0');
      |     end
      |   else
      |     tmps=num2str(fltCC2sc_D);
      |     if ~strcmp(fltCC2sc_D_bkup,tmps)
      |       set_param(gcb,'fltCC2sc_D',tmps);
      |     end
      |   end
      |   if isnan(fltCC1sc_Q)
      |     if ~strcmp(fltCC1sc_Q_bkup,'0')
      |       set_param(gcb,'fltCC1sc_Q','0');
      |     end
      |   else
      |     tmps=num2str(fltCC1sc_Q);
      |     if ~strcmp(fltCC1sc_Q_bkup,tmps)
      |       set_param(gcb,'fltCC1sc_Q',tmps);
      |     end
      |   end
      |   if isnan(fltCC2sc_Q)
      |     if ~strcmp(fltCC2sc_Q_bkup,'0')
      |       set_param(gcb,'fltCC2sc_Q','0');
      |     end
      |   else
      |     tmps=num2str(fltCC2sc_Q);
      |     if ~strcmp(fltCC2sc_Q_bkup,tmps)
      |       set_param(gcb,'fltCC2sc_Q',tmps);
      |     end
      |   end
      | end
      mask Callback Ld:
      | autoCalcEn=get_param(gcb,'autoCalcEn');
      | if strcmp(autoCalcEn,'on')
      |   SampleTime=Simulink.data.evalinGlobal(bdroot,get_param(gcb,'SampleTime'));
      |   if (SampleTime==-1)
      |     SampleTime=str2double(get_param(gcb,'SampleTime_1'));
      |   end
      |   fltCC1sc_D_bkup=get_param(gcb,'fltCC1sc_D');
      |   fltCC2sc_D_bkup=get_param(gcb,'fltCC2sc_D');
      |   fltCC1sc_Q_bkup=get_param(gcb,'fltCC1sc_Q');
      |   fltCC2sc_Q_bkup=get_param(gcb,'fltCC2sc_Q');
      |   intmethod=get_param(gcb,'intmethod');
      |   if0=Simulink.data.evalinGlobal(bdroot,get_param(gcb,'if0'));
      |   iksi=Simulink.data.evalinGlobal(bdroot,get_param(gcb,'iksi'));
      |   Ld=Simulink.data.evalinGlobal(bdroot,get_param(gcb,'Ld'));
      |   Lq=Simulink.data.evalinGlobal(bdroot,get_param(gcb,'Lq'));
      |   Rs=Simulink.data.evalinGlobal(bdroot,get_param(gcb,'Rs'));
      |   if (if0<=0)
      |     warning('Natural frequency f0 must be positive.');
      |   end
      |   if (iksi<=0)
      |     warning('Current loop attenuation must be positive.');
      |   end
      |   if (iksi>1)
      |     warning('Current loop attenuation must not exceed 1.');
      |   end
      |   if (Ld<=0)
      |     warning('Inductance Ld must be positive.');
      |   end
      |   if (Lq<=0)
      |     warning('Inductance Lq must be positive.');
      |   end
      |   if (Rs<0)
      |     warning('Resistance Rs must be non-negative.');
      |   end
      |   w0=6.283185307179586*if0;
      |   pgainD=2.0*iksi*w0*Ld-Rs;
      |   igainD=w0*w0*Ld;
      |   pgainQ=2.0*iksi*w0*Lq-Rs;
      |   igainQ=w0*w0*Lq;
      |   if strcmp(intmethod,'Forward Rectangular')
      |     cc1d=pgainD;
      |     cc2d=-pgainD+igainD*SampleTime;
      |     cc1q=pgainQ;
      |     cc2q=-pgainQ+igainQ*SampleTime;
      |   else
      |     if strcmp(intmethod,'Backward Rectangular')
      |       cc1d=pgainD+igainD*SampleTime;
      |       cc2d=-pgainD;
      |       cc1q=pgainQ+igainQ*SampleTime;
      |       cc2q=-pgainQ;
      |     else
      |       cc1d=pgainD+igainD*SampleTime*0.5;
      |       cc2d=-pgainD+igainD*SampleTime*0.5;
      |       cc1q=pgainQ+igainQ*SampleTime*0.5;
      |       cc2q=-pgainQ+igainQ*SampleTime*0.5;
      |     end
      |   end
      |   fltCC1sc_D=cc1d;
      |   fltCC2sc_D=cc2d;
      |   fltCC1sc_Q=cc1q;
      |   fltCC2sc_Q=cc2q;
      |   if isnan(fltCC1sc_D)
      |     if ~strcmp(fltCC1sc_D_bkup,'0')
      |       set_param(gcb,'fltCC1sc_D','0');
      |     end
      |   else
      |     tmps=num2str(fltCC1sc_D);
      |     if ~strcmp(fltCC1sc_D_bkup,tmps)
      |       set_param(gcb,'fltCC1sc_D',tmps);
      |     end
      |   end
      |   if isnan(fltCC2sc_D)
      |     if ~strcmp(fltCC2sc_D_bkup,'0')
      |       set_param(gcb,'fltCC2sc_D','0');
      |     end
      |   else
      |     tmps=num2str(fltCC2sc_D);
      |     if ~strcmp(fltCC2sc_D_bkup,tmps)
      |       set_param(gcb,'fltCC2sc_D',tmps);
      |     end
      |   end
      |   if isnan(fltCC1sc_Q)
      |     if ~strcmp(fltCC1sc_Q_bkup,'0')
      |       set_param(gcb,'fltCC1sc_Q','0');
      |     end
      |   else
      |     tmps=num2str(fltCC1sc_Q);
      |     if ~strcmp(fltCC1sc_Q_bkup,tmps)
      |       set_param(gcb,'fltCC1sc_Q',tmps);
      |     end
      |   end
      |   if isnan(fltCC2sc_Q)
      |     if ~strcmp(fltCC2sc_Q_bkup,'0')
      |       set_param(gcb,'fltCC2sc_Q','0');
      |     end
      |   else
      |     tmps=num2str(fltCC2sc_Q);
      |     if ~strcmp(fltCC2sc_Q_bkup,tmps)
      |       set_param(gcb,'fltCC2sc_Q',tmps);
      |     end
      |   end
      | end
      mask Callback Lq:
      | autoCalcEn=get_param(gcb,'autoCalcEn');
      | if strcmp(autoCalcEn,'on')
      |   SampleTime=Simulink.data.evalinGlobal(bdroot,get_param(gcb,'SampleTime'));
      |   if (SampleTime==-1)
      |     SampleTime=str2double(get_param(gcb,'SampleTime_1'));
      |   end
      |   fltCC1sc_D_bkup=get_param(gcb,'fltCC1sc_D');
      |   fltCC2sc_D_bkup=get_param(gcb,'fltCC2sc_D');
      |   fltCC1sc_Q_bkup=get_param(gcb,'fltCC1sc_Q');
      |   fltCC2sc_Q_bkup=get_param(gcb,'fltCC2sc_Q');
      |   intmethod=get_param(gcb,'intmethod');
      |   if0=Simulink.data.evalinGlobal(bdroot,get_param(gcb,'if0'));
      |   iksi=Simulink.data.evalinGlobal(bdroot,get_param(gcb,'iksi'));
      |   Ld=Simulink.data.evalinGlobal(bdroot,get_param(gcb,'Ld'));
      |   Lq=Simulink.data.evalinGlobal(bdroot,get_param(gcb,'Lq'));
      |   Rs=Simulink.data.evalinGlobal(bdroot,get_param(gcb,'Rs'));
      |   if (if0<=0)
      |     warning('Natural frequency f0 must be positive.');
      |   end
      |   if (iksi<=0)
      |     warning('Current loop attenuation must be positive.');
      |   end
      |   if (iksi>1)
      |     warning('Current loop attenuation must not exceed 1.');
      |   end
      |   if (Ld<=0)
      |     warning('Inductance Ld must be positive.');
      |   end
      |   if (Lq<=0)
      |     warning('Inductance Lq must be positive.');
      |   end
      |   if (Rs<0)
      |     warning('Resistance Rs must be non-negative.');
      |   end
      |   w0=6.283185307179586*if0;
      |   pgainD=2.0*iksi*w0*Ld-Rs;
      |   igainD=w0*w0*Ld;
      |   pgainQ=2.0*iksi*w0*Lq-Rs;
      |   igainQ=w0*w0*Lq;
      |   if strcmp(intmethod,'Forward Rectangular')
      |     cc1d=pgainD;
      |     cc2d=-pgainD+igainD*SampleTime;
      |     cc1q=pgainQ;
      |     cc2q=-pgainQ+igainQ*SampleTime;
      |   else
      |     if strcmp(intmethod,'Backward Rectangular')
      |       cc1d=pgainD+igainD*SampleTime;
      |       cc2d=-pgainD;
      |       cc1q=pgainQ+igainQ*SampleTime;
      |       cc2q=-pgainQ;
      |     else
      |       cc1d=pgainD+igainD*SampleTime*0.5;
      |       cc2d=-pgainD+igainD*SampleTime*0.5;
      |       cc1q=pgainQ+igainQ*SampleTime*0.5;
      |       cc2q=-pgainQ+igainQ*SampleTime*0.5;
      |     end
      |   end
      |   fltCC1sc_D=cc1d;
      |   fltCC2sc_D=cc2d;
      |   fltCC1sc_Q=cc1q;
      |   fltCC2sc_Q=cc2q;
      |   if isnan(fltCC1sc_D)
      |     if ~strcmp(fltCC1sc_D_bkup,'0')
      |       set_param(gcb,'fltCC1sc_D','0');
      |     end
      |   else
      |     tmps=num2str(fltCC1sc_D);
      |     if ~strcmp(fltCC1sc_D_bkup,tmps)
      |       set_param(gcb,'fltCC1sc_D',tmps);
      |     end
      |   end
      |   if isnan(fltCC2sc_D)
      |     if ~strcmp(fltCC2sc_D_bkup,'0')
      |       set_param(gcb,'fltCC2sc_D','0');
      |     end
      |   else
      |     tmps=num2str(fltCC2sc_D);
      |     if ~strcmp(fltCC2sc_D_bkup,tmps)
      |       set_param(gcb,'fltCC2sc_D',tmps);
      |     end
      |   end
      |   if isnan(fltCC1sc_Q)
      |     if ~strcmp(fltCC1sc_Q_bkup,'0')
      |       set_param(gcb,'fltCC1sc_Q','0');
      |     end
      |   else
      |     tmps=num2str(fltCC1sc_Q);
      |     if ~strcmp(fltCC1sc_Q_bkup,tmps)
      |       set_param(gcb,'fltCC1sc_Q',tmps);
      |     end
      |   end
      |   if isnan(fltCC2sc_Q)
      |     if ~strcmp(fltCC2sc_Q_bkup,'0')
      |       set_param(gcb,'fltCC2sc_Q','0');
      |     end
      |   else
      |     tmps=num2str(fltCC2sc_Q);
      |     if ~strcmp(fltCC2sc_Q_bkup,tmps)
      |       set_param(gcb,'fltCC2sc_Q',tmps);
      |     end
      |   end
      | end
      mask Callback Rs:
      | autoCalcEn=get_param(gcb,'autoCalcEn');
      | if strcmp(autoCalcEn,'on')
      |   SampleTime=Simulink.data.evalinGlobal(bdroot,get_param(gcb,'SampleTime'));
      |   if (SampleTime==-1)
      |     SampleTime=str2double(get_param(gcb,'SampleTime_1'));
      |   end
      |   fltCC1sc_D_bkup=get_param(gcb,'fltCC1sc_D');
      |   fltCC2sc_D_bkup=get_param(gcb,'fltCC2sc_D');
      |   fltCC1sc_Q_bkup=get_param(gcb,'fltCC1sc_Q');
      |   fltCC2sc_Q_bkup=get_param(gcb,'fltCC2sc_Q');
      |   intmethod=get_param(gcb,'intmethod');
      |   if0=Simulink.data.evalinGlobal(bdroot,get_param(gcb,'if0'));
      |   iksi=Simulink.data.evalinGlobal(bdroot,get_param(gcb,'iksi'));
      |   Ld=Simulink.data.evalinGlobal(bdroot,get_param(gcb,'Ld'));
      |   Lq=Simulink.data.evalinGlobal(bdroot,get_param(gcb,'Lq'));
      |   Rs=Simulink.data.evalinGlobal(bdroot,get_param(gcb,'Rs'));
      |   if (if0<=0)
      |     warning('Natural frequency f0 must be positive.');
      |   end
      |   if (iksi<=0)
      |     warning('Current loop attenuation must be positive.');
      |   end
      |   if (iksi>1)
      |     warning('Current loop attenuation must not exceed 1.');
      |   end
      |   if (Ld<=0)
      |     warning('Inductance Ld must be positive.');
      |   end
      |   if (Lq<=0)
      |     warning('Inductance Lq must be positive.');
      |   end
      |   if (Rs<0)
      |     warning('Resistance Rs must be non-negative.');
      |   end
      |   w0=6.283185307179586*if0;
      |   pgainD=2.0*iksi*w0*Ld-Rs;
      |   igainD=w0*w0*Ld;
      |   pgainQ=2.0*iksi*w0*Lq-Rs;
      |   igainQ=w0*w0*Lq;
      |   if strcmp(intmethod,'Forward Rectangular')
      |     cc1d=pgainD;
      |     cc2d=-pgainD+igainD*SampleTime;
      |     cc1q=pgainQ;
      |     cc2q=-pgainQ+igainQ*SampleTime;
      |   else
      |     if strcmp(intmethod,'Backward Rectangular')
      |       cc1d=pgainD+igainD*SampleTime;
      |       cc2d=-pgainD;
      |       cc1q=pgainQ+igainQ*SampleTime;
      |       cc2q=-pgainQ;
      |     else
      |       cc1d=pgainD+igainD*SampleTime*0.5;
      |       cc2d=-pgainD+igainD*SampleTime*0.5;
      |       cc1q=pgainQ+igainQ*SampleTime*0.5;
      |       cc2q=-pgainQ+igainQ*SampleTime*0.5;
      |     end
      |   end
      |   fltCC1sc_D=cc1d;
      |   fltCC2sc_D=cc2d;
      |   fltCC1sc_Q=cc1q;
      |   fltCC2sc_Q=cc2q;
      |   if isnan(fltCC1sc_D)
      |     if ~strcmp(fltCC1sc_D_bkup,'0')
      |       set_param(gcb,'fltCC1sc_D','0');
      |     end
      |   else
      |     tmps=num2str(fltCC1sc_D);
      |     if ~strcmp(fltCC1sc_D_bkup,tmps)
      |       set_param(gcb,'fltCC1sc_D',tmps);
      |     end
      |   end
      |   if isnan(fltCC2sc_D)
      |     if ~strcmp(fltCC2sc_D_bkup,'0')
      |       set_param(gcb,'fltCC2sc_D','0');
      |     end
      |   else
      |     tmps=num2str(fltCC2sc_D);
      |     if ~strcmp(fltCC2sc_D_bkup,tmps)
      |       set_param(gcb,'fltCC2sc_D',tmps);
      |     end
      |   end
      |   if isnan(fltCC1sc_Q)
      |     if ~strcmp(fltCC1sc_Q_bkup,'0')
      |       set_param(gcb,'fltCC1sc_Q','0');
      |     end
      |   else
      |     tmps=num2str(fltCC1sc_Q);
      |     if ~strcmp(fltCC1sc_Q_bkup,tmps)
      |       set_param(gcb,'fltCC1sc_Q',tmps);
      |     end
      |   end
      |   if isnan(fltCC2sc_Q)
      |     if ~strcmp(fltCC2sc_Q_bkup,'0')
      |       set_param(gcb,'fltCC2sc_Q','0');
      |     end
      |   else
      |     tmps=num2str(fltCC2sc_Q);
      |     if ~strcmp(fltCC2sc_Q_bkup,tmps)
      |       set_param(gcb,'fltCC2sc_Q',tmps);
      |     end
      |   end
      | end
      mask Callback autoCalcEn:
      | maskStr=get_param(gcb,'showStates');
      | if strcmp(maskStr,'Hide (faster execution)')
      |   p=Simulink.Mask.get(gcb);
      |   autoCalcEn=get_param(gcb,'autoCalcEn');
      |   hintText=p.getDialogControl('timeHint');
      |   if strcmp(autoCalcEn,'on')
      |     param=p.getParameter('Rs');
      |     if strcmp(param.Enabled,'off')
      |       SampleTime=Simulink.data.evalinGlobal(bdroot,get_param(gcb,'SampleTime'));
      |       if SampleTime==-1
      |         SampleTime=str2double(get_param(gcb,'SampleTime_1'));
      |         if isnan(SampleTime)
      |           hintText.Prompt=['Note: Implementation parameters cannot be calculated yet because the block''s inherited sample time is unknown. Simulink will update the sample time when you run the simulation.'];
      |         else
      |           hintText.Prompt=['Caution: Implementation parameters depend on inherited sample time. Make sure that the sample time of the block''s inputs corresponds to the sampling period in the target application.'];
      |         end
      |       else
      |         hintText.Prompt='Caution: Implementation parameters depend on the sample time. Make sure that the simulation time step corresponds to the sampling period in the target application.';
      |       end
      |       p=Simulink.Mask.get(gcb);
      |       param=p.getParameter('intmethod');
      |       param.set('Enabled','on');
      |       param=p.getParameter('if0');
      |       param.set('Enabled','on');
      |       param=p.getParameter('iksi');
      |       param.set('Enabled','on');
      |       param=p.getParameter('Ld');
      |       param.set('Enabled','on');
      |       param=p.getParameter('Lq');
      |       param.set('Enabled','on');
      |       param=p.getParameter('Rs');
      |       param.set('Enabled','on');
      |     else
      |       SampleTime=Simulink.data.evalinGlobal(bdroot,get_param(gcb,'SampleTime'));
      |       if SampleTime==-1
      |         SampleTime=str2double(get_param(gcb,'SampleTime_1'));
      |       end
      |     end
      |     fltCC1sc_D_bkup=get_param(gcb,'fltCC1sc_D');
      |     fltCC2sc_D_bkup=get_param(gcb,'fltCC2sc_D');
      |     fltCC1sc_Q_bkup=get_param(gcb,'fltCC1sc_Q');
      |     fltCC2sc_Q_bkup=get_param(gcb,'fltCC2sc_Q');
      |     intmethod=get_param(gcb,'intmethod');
      |     if0=Simulink.data.evalinGlobal(bdroot,get_param(gcb,'if0'));
      |     iksi=Simulink.data.evalinGlobal(bdroot,get_param(gcb,'iksi'));
      |     Ld=Simulink.data.evalinGlobal(bdroot,get_param(gcb,'Ld'));
      |     Lq=Simulink.data.evalinGlobal(bdroot,get_param(gcb,'Lq'));
      |     Rs=Simulink.data.evalinGlobal(bdroot,get_param(gcb,'Rs'));
      |     if (if0<=0)
      |       warning('Natural frequency f0 must be positive.');
      |     end
      |     if (iksi<=0)
      |       warning('Current loop attenuation must be positive.');
      |     end
      |     if (iksi>1)
      |       warning('Current loop attenuation must not exceed 1.');
      |     end
      |     if (Ld<=0)
      |       warning('Inductance Ld must be positive.');
      |     end
      |     if (Lq<=0)
      |       warning('Inductance Lq must be positive.');
      |     end
      |     if (Rs<0)
      |       warning('Resistance Rs must be non-negative.');
      |     end
      |     w0=6.283185307179586*if0;
      |     pgainD=2.0*iksi*w0*Ld-Rs;
      |     igainD=w0*w0*Ld;
      |     pgainQ=2.0*iksi*w0*Lq-Rs;
      |     igainQ=w0*w0*Lq;
      |     if strcmp(intmethod,'Forward Rectangular')
      |       cc1d=pgainD;
      |       cc2d=-pgainD+igainD*SampleTime;
      |       cc1q=pgainQ;
      |       cc2q=-pgainQ+igainQ*SampleTime;
      |     else
      |       if strcmp(intmethod,'Backward Rectangular')
      |         cc1d=pgainD+igainD*SampleTime;
      |         cc2d=-pgainD;
      |         cc1q=pgainQ+igainQ*SampleTime;
      |         cc2q=-pgainQ;
      |       else
      |         cc1d=pgainD+igainD*SampleTime*0.5;
      |         cc2d=-pgainD+igainD*SampleTime*0.5;
      |         cc1q=pgainQ+igainQ*SampleTime*0.5;
      |         cc2q=-pgainQ+igainQ*SampleTime*0.5;
      |       end
      |     end
      |     fltCC1sc_D=cc1d;
      |     fltCC2sc_D=cc2d;
      |     fltCC1sc_Q=cc1q;
      |     fltCC2sc_Q=cc2q;
      |     if isnan(fltCC1sc_D)
      |       if ~strcmp(fltCC1sc_D_bkup,'0')
      |         set_param(gcb,'fltCC1sc_D','0');
      |       end
      |     else
      |       tmps=num2str(fltCC1sc_D);
      |       if ~strcmp(fltCC1sc_D_bkup,tmps)
      |         set_param(gcb,'fltCC1sc_D',tmps);
      |       end
      |     end
      |     if isnan(fltCC2sc_D)
      |       if ~strcmp(fltCC2sc_D_bkup,'0')
      |         set_param(gcb,'fltCC2sc_D','0');
      |       end
      |     else
      |       tmps=num2str(fltCC2sc_D);
      |       if ~strcmp(fltCC2sc_D_bkup,tmps)
      |         set_param(gcb,'fltCC2sc_D',tmps);
      |       end
      |     end
      |     if isnan(fltCC1sc_Q)
      |       if ~strcmp(fltCC1sc_Q_bkup,'0')
      |         set_param(gcb,'fltCC1sc_Q','0');
      |       end
      |     else
      |       tmps=num2str(fltCC1sc_Q);
      |       if ~strcmp(fltCC1sc_Q_bkup,tmps)
      |         set_param(gcb,'fltCC1sc_Q',tmps);
      |       end
      |     end
      |     if isnan(fltCC2sc_Q)
      |       if ~strcmp(fltCC2sc_Q_bkup,'0')
      |         set_param(gcb,'fltCC2sc_Q','0');
      |       end
      |     else
      |       tmps=num2str(fltCC2sc_Q);
      |       if ~strcmp(fltCC2sc_Q_bkup,tmps)
      |         set_param(gcb,'fltCC2sc_Q',tmps);
      |       end
      |     end
      |   else
      |     param=p.getParameter('Rs');
      |     if strcmp(param.Enabled,'on')
      |       hintText.Prompt='Caution: Implementation parameters are fixed.';
      |       p=Simulink.Mask.get(gcb);
      |       param=p.getParameter('intmethod');
      |       param.set('Enabled','off');
      |       param=p.getParameter('if0');
      |       param.set('Enabled','off');
      |       param=p.getParameter('iksi');
      |       param.set('Enabled','off');
      |       param=p.getParameter('Ld');
      |       param.set('Enabled','off');
      |       param=p.getParameter('Lq');
      |       param.set('Enabled','off');
      |       param=p.getParameter('Rs');
      |       param.set('Enabled','off');
      |     end
      |   end
      | end
      mask DialogControl CompBut Prompt: Recalculate sample times
      mask DialogControl CompBut Tooltip: Simulink updates the sample times of all blocks when the simulation is run. This button will update the sample times now.
      mask DialogControl CompBut Callback:
      | btn=questdlg('This will apply all changes in all open dialog boxes and update the schematic. Do you want to proceed?','Apply all changes','Continue','Cancel','Continue');
      | if strcmp(btn,'Continue')
      |   dlgs=DAStudio.ToolRoot.getOpenDialogs;
      |   for i=1:length(dlgs)
      |     dlgs(i).apply;
      |   end
      |   try
      |     SampleTime_1=str2double(get_param(gcb,'SampleTime_1'));
      |     ts=Simulink.Block.getSampleTimes(gcb);
      |     ts=ts(1).Value(1);
      |     if (SampleTime_1 ~= ts)
      |       SampleTime_1=ts;
      |       set_param(gcb,'SampleTime_1',num2str(ts));
      |       autoCalcEn=get_param(gcb,'autoCalcEn');
      |       if strcmp(autoCalcEn,'on')
      |         SampleTime=Simulink.data.evalinGlobal(bdroot,get_param(gcb,'SampleTime'));
      |         p=Simulink.Mask.get(gcb);
      |         hintText=p.getDialogControl('timeHint');
      |         if SampleTime==-1
      |           SampleTime=SampleTime_1;
      |           hintText.Prompt='Caution: Implementation parameters depend on inherited sample time. Make sure that the sample time of the block''s inputs corresponds to the sampling period in the target application.';
      |         else
      |           hintText.Prompt='Caution: Implementation parameters depend on the sample time. Make sure that the simulation time step corresponds to the sampling period in the target application.';
      |         end
      |         fltCC1sc_D_bkup=get_param(gcb,'fltCC1sc_D');
      |         fltCC2sc_D_bkup=get_param(gcb,'fltCC2sc_D');
      |         fltCC1sc_Q_bkup=get_param(gcb,'fltCC1sc_Q');
      |         fltCC2sc_Q_bkup=get_param(gcb,'fltCC2sc_Q');
      |         intmethod=get_param(gcb,'intmethod');
      |         if0=Simulink.data.evalinGlobal(bdroot,get_param(gcb,'if0'));
      |         iksi=Simulink.data.evalinGlobal(bdroot,get_param(gcb,'iksi'));
      |         Ld=Simulink.data.evalinGlobal(bdroot,get_param(gcb,'Ld'));
      |         Lq=Simulink.data.evalinGlobal(bdroot,get_param(gcb,'Lq'));
      |         Rs=Simulink.data.evalinGlobal(bdroot,get_param(gcb,'Rs'));
      |         if (if0<=0)
      |           warning('Natural frequency f0 must be positive.');
      |         end
      |         if (iksi<=0)
      |           warning('Current loop attenuation must be positive.');
      |         end
      |         if (iksi>1)
      |           warning('Current loop attenuation must not exceed 1.');
      |         end
      |         if (Ld<=0)
      |           warning('Inductance Ld must be positive.');
      |         end
      |         if (Lq<=0)
      |           warning('Inductance Lq must be positive.');
      |         end
      |         if (Rs<0)
      |           warning('Resistance Rs must be non-negative.');
      |         end
      |         w0=6.283185307179586*if0;
      |         pgainD=2.0*iksi*w0*Ld-Rs;
      |         igainD=w0*w0*Ld;
      |         pgainQ=2.0*iksi*w0*Lq-Rs;
      |         igainQ=w0*w0*Lq;
      |         if strcmp(intmethod,'Forward Rectangular')
      |           cc1d=pgainD;
      |           cc2d=-pgainD+igainD*SampleTime;
      |           cc1q=pgainQ;
      |           cc2q=-pgainQ+igainQ*SampleTime;
      |         else
      |           if strcmp(intmethod,'Backward Rectangular')
      |             cc1d=pgainD+igainD*SampleTime;
      |             cc2d=-pgainD;
      |             cc1q=pgainQ+igainQ*SampleTime;
      |             cc2q=-pgainQ;
      |           else
      |             cc1d=pgainD+igainD*SampleTime*0.5;
      |             cc2d=-pgainD+igainD*SampleTime*0.5;
      |             cc1q=pgainQ+igainQ*SampleTime*0.5;
      |             cc2q=-pgainQ+igainQ*SampleTime*0.5;
      |           end
      |         end
      |         fltCC1sc_D=cc1d;
      |         fltCC2sc_D=cc2d;
      |         fltCC1sc_Q=cc1q;
      |         fltCC2sc_Q=cc2q;
      |         if isnan(fltCC1sc_D)
      |           if ~strcmp(fltCC1sc_D_bkup,'0')
      |             set_param(gcb,'fltCC1sc_D','0');
      |           end
      |         else
      |           tmps=num2str(fltCC1sc_D);
      |           if ~strcmp(fltCC1sc_D_bkup,tmps)
      |             set_param(gcb,'fltCC1sc_D',tmps);
      |           end
      |         end
      |         if isnan(fltCC2sc_D)
      |           if ~strcmp(fltCC2sc_D_bkup,'0')
      |             set_param(gcb,'fltCC2sc_D','0');
      |           end
      |         else
      |           tmps=num2str(fltCC2sc_D);
      |           if ~strcmp(fltCC2sc_D_bkup,tmps)
      |             set_param(gcb,'fltCC2sc_D',tmps);
      |           end
      |         end
      |         if isnan(fltCC1sc_Q)
      |           if ~strcmp(fltCC1sc_Q_bkup,'0')
      |             set_param(gcb,'fltCC1sc_Q','0');
      |           end
      |         else
      |           tmps=num2str(fltCC1sc_Q);
      |           if ~strcmp(fltCC1sc_Q_bkup,tmps)
      |             set_param(gcb,'fltCC1sc_Q',tmps);
      |           end
      |         end
      |         if isnan(fltCC2sc_Q)
      |           if ~strcmp(fltCC2sc_Q_bkup,'0')
      |             set_param(gcb,'fltCC2sc_Q','0');
      |           end
      |         else
      |           tmps=num2str(fltCC2sc_Q);
      |           if ~strcmp(fltCC2sc_Q_bkup,tmps)
      |             set_param(gcb,'fltCC2sc_Q',tmps);
      |           end
      |         end
      |       end
      |     end
      |   catch
      |    warning(['Sample time cannot be calculated for the block ' gcb])
      |   end
      | end
      mask DialogControl timeHint Prompt: Note: Implementation parameters cannot be calculated yet because the block's inherited sample time is unknown. Simulink will update the sample time when you run the simulation.
      mask Display:
      | color('black');
      | pos = get_param(gcb, 'Position');
      | width = pos(3) - pos(1);
      | height = pos(4) - pos(2);
      | tX=width/2;
      | tY=height - 25;
      | color('black');
      | text(tX,tY, 'AMCLIB_CurrentLoop_FLT', 'horizontalAlignment', 'center');
      | if showStates == 2
      |   color('red');
      |   text(tX,tY - 20, ['debugging mode' char(13) char(10) '(limited performance)'], 'horizontalAlignment', 'center');
      | end
  AMCLIB_EstimBJ_FLT : Subsystem  TreatAsAtomicUnit=on  mask(AMCLIB_EstimBJ_FLT){cfg=Basic, u32SamplingFreq=10000, fltIN=5, fltWN=3000, fltPP=3, fltLd=0.00022, fltLq=0.00027, fltRs=0.376, fltDtVDrop=0.164333, fltAlignTime=0, fltIReqOl=0, fltWStepOl=0, fltDCWReq1=0, fltDCWReq2=0, fltDcPiPropGain=0, fltDcPiIntegGain=0, fltAcPiPropGain=0, fltAcPiIntegGain=0}
      mask prompts: cfg "Configuration preset:"
      mask help: PMSM mechanical parameters estimator in single precision floating-point implementation. Refer to the AMMCLIB User's Guide for further details.
      mask init:
      | ddName = get_param(bdroot,'DataDictionary');
      | if length(ddName)==0
      |   set_param(bdroot,'DataDictionary','ammclib_types.sldd');
      | else
      |   dd = Simulink.data.dictionary.open(ddName);
      |   data = getSection(dd,'Design Data');
      |   if ~exist(data,'SWLIBS_2Syst_F16')
      |     addDataSource(dd,'ammclib_types.sldd');
      |     saveChanges(dd);
      |   end
      | end
      | posblk = get_param(gcb, 'Position');
      settings: RTWSystemCode=Inline
      mask Help: web([fileparts(which('ammclib_bam_S32K3xx.slx')) '/../doc/S32K3XXMCLUG.pdf'], '-browser')
      mask TypeOptions cfg: Basic | Advanced
      mask Callback cfg:
      | maskStr = get_param(gcb,'cfg');
      | if strcmp(maskStr,'Basic')
      |   set_param(gcb,'MaskEnables',{'on','on','on','on','on','on','on','on','on','off','off','off','off','off','off','off','off','off'});
      | end
      | if strcmp(maskStr,'Advanced')
      |   set_param(gcb,'MaskEnables',{'on','on','on','on','on','on','on','on','on','on','on','on','on','on','on','on','on','on'});
      | end
      mask Display: pos = get_param(gcb, 'Position');width = pos(3) - pos(1); height = pos(4) - pos(2);tX=width/2;tY=height - 8;color('black');text(tX,tY, 'AMCLIB_EstimBJ_FLT', 'horizontalAlignment', 'center');
  AMCLIB_EstimRL_FLT : Subsystem  TreatAsAtomicUnit=on  mask(AMCLIB_EstimRL_FLT){u32SamplingFreq=10000, fltIDcMax=10, u16LdqNumMeas=5, fltIDcLd=0, fltIDcLq=0, fltIDcNegMax=0, cfg=DEFAULT}
      mask prompts: u32SamplingFreq "u32SamplingFreq (Sampling frequency of the control loop [Hz]):"; fltIDcMax "fltIDcMax (maximal DC current or motor nominal current [A]):"; u16LdqNumMeas "u16LdqNumMeas (Number of DC current steps used for
the measurement of electrical parameters):"; fltIDcLd "fltIDcLd (DC current used for Ld measurement [A]):"; fltIDcLq "fltIDcLq (DC current used for Lq measurement [A]):"; fltIDcNegMax "fltIDcNegMax (Largest allowed negative DC current [A]):"; cfg "Configuration preset:"
      mask help: PMSM electrical parameters estimator in single precision floating-point implementation. Refer to the AMMCLIB User's Guide for further details.
      mask init:
      | ddName = get_param(bdroot,'DataDictionary');
      | if length(ddName)==0
      |   set_param(bdroot,'DataDictionary','ammclib_types.sldd');
      | else
      |   dd = Simulink.data.dictionary.open(ddName);
      |   data = getSection(dd,'Design Data');
      |   if ~exist(data,'SWLIBS_2Syst_F16')
      |     addDataSource(dd,'ammclib_types.sldd');
      |     saveChanges(dd);
      |   end
      | end
      | posblk = get_param(gcb, 'Position');
      | 
      | if (cfg == 1) || (cfg == 2) || (cfg == 3)
      |   if strcmp(get_param([gcb '/fltIDcDReq'], 'BlockType'), 'Inport')
      |     if strcmp(get_param([gcb '/fltIDcDReq'], 'BlockType'), 'Inport')
      |       pos = get_param([gcb, '/fltIDcDReq'], 'Position');
      |       orient = get_param([gcb, '/fltIDcDReq'], 'Orientation');
      |       delete_block([gcb, '/fltIDcDReq']);
      |       add_block('built-in/Ground', [gcb, '/fltIDcDReq'], 'Position', pos, 'Orientation', orient);
      |     end
      | 
      |     if strcmp(get_param([gcb '/fltIDcQReq'], 'BlockType'), 'Inport')
      |       pos = get_param([gcb, '/fltIDcQReq'], 'Position');
      |       orient = get_param([gcb, '/fltIDcQReq'], 'Orientation');
      |       delete_block([gcb, '/fltIDcQReq']);
      |       add_block('built-in/Ground', [gcb, '/fltIDcQReq'], 'Position', pos, 'Orientation', orient);
      |     end
      | 
      |     if strcmp(get_param([gcb '/fltIAcReq'], 'BlockType'), 'Inport')
      |       pos = get_param([gcb, '/fltIAcReq'], 'Position');
      |       orient = get_param([gcb, '/fltIAcReq'], 'Orientation');
      |       delete_block([gcb, '/fltIAcReq']);
      |       add_block('built-in/Ground', [gcb, '/fltIAcReq'], 'Position', pos, 'Orientation', orient);
      |     end
      | 
      |     if strcmp(get_param([gcb '/u16FAc'], 'BlockType'), 'Inport')
      |       pos = get_param([gcb, '/u16FAc'], 'Position');
      |       orient = get_param([gcb, '/u16FAc'], 'Orientation');
      |       delete_block([gcb, '/u16FAc']);
      |       add_block('built-in/Ground', [gcb, '/u16FAc'], 'Position', pos, 'Orientation', orient);
      |     end
      | 
      |     if strcmp(get_param([gcb '/u8LdqSwitch'], 'BlockType'), 'Inport')
      |       pos = get_param([gcb, '/u8LdqSwitch'], 'Position');
      |       orient = get_param([gcb, '/u8LdqSwitch'], 'Orientation');
      |       delete_block([gcb, '/u8LdqSwitch']);
      |       add_block('built-in/Ground', [gcb, '/u8LdqSwitch'], 'Position', pos, 'Orientation', orient);
      |     end
      | 
      |     set_param([gcb '/pIAlBeFbck'], 'Port', '1');
      |     set_param([gcb '/fltUDcBus'], 'Port', '2');
      | 
      | 
      |     if (posblk(4) - posblk(2)) < 200
      |       height = 200;
      |       set_param(gcb,'Position',[posblk(1), posblk(2), posblk(3), posblk(2)+height])
      |     end
      |   end
      | end
      | if (cfg == 4)
      |   if strcmp(get_param([gcb '/fltIDcDReq'], 'BlockType'), 'Ground')
      |     if strcmp(get_param([gcb '/fltIDcDReq'], 'BlockType'), 'Ground')
      |       pos = get_param([gcb, '/fltIDcDReq'], 'Position');
      |       orient = get_param([gcb, '/fltIDcDReq'], 'Orientation');
      |       delete_block([gcb, '/fltIDcDReq']);
      |       add_block('built-in/Inport', [gcb, '/fltIDcDReq'], 'Position', pos, 'Orientation', orient, 'OutDataTypeStr', 'single');
      |     end
      | 
      |     if strcmp(get_param([gcb '/fltIDcQReq'], 'BlockType'), 'Ground')
      |       pos = get_param([gcb, '/fltIDcQReq'], 'Position');
      |       orient = get_param([gcb, '/fltIDcQReq'], 'Orientation');
      |       delete_block([gcb, '/fltIDcQReq']);
      |       add_block('built-in/Inport', [gcb, '/fltIDcQReq'], 'Position', pos, 'Orientation', orient, 'OutDataTypeStr', 'single');
      |     end
      | 
      |     if strcmp(get_param([gcb '/fltIAcReq'], 'BlockType'), 'Ground')
      |       pos = get_param([gcb, '/fltIAcReq'], 'Position');
      |       orient = get_param([gcb, '/fltIAcReq'], 'Orientation');
      |       delete_block([gcb, '/fltIAcReq']);
      |       add_block('built-in/Inport', [gcb, '/fltIAcReq'], 'Position', pos, 'Orientation', orient, 'OutDataTypeStr', 'single');
      |     end
      | 
      |     if strcmp(get_param([gcb '/u16FAc'], 'BlockType'), 'Ground')
      |       pos = get_param([gcb, '/u16FAc'], 'Position');
      |       orient = get_param([gcb, '/u16FAc'], 'Orientation');
      |       delete_block([gcb, '/u16FAc']);
      |       add_block('built-in/Inport', [gcb, '/u16FAc'], 'Position', pos, 'Orientation', orient, 'OutDataTypeStr', 'uint16');
      |     end
      | 
      |     if strcmp(get_param([gcb '/u8LdqSwitch'], 'BlockType'), 'Ground')
      |       pos = get_param([gcb, '/u8LdqSwitch'], 'Position');
      |       orient = get_param([gcb, '/u8LdqSwitch'], 'Orientation');
      |       delete_block([gcb, '/u8LdqSwitch']);
      |       add_block('built-in/Inport', [gcb, '/u8LdqSwitch'], 'Position', pos, 'Orientation', orient, 'OutDataTypeStr', 'uint8');
      |     end
      | 
      |     set_param([gcb '/pIAlBeFbck'], 'Port', '1');
      |     set_param([gcb '/fltUDcBus'], 'Port', '2');
      |     set_param([gcb '/fltIDcDReq'], 'Port', '3');
      |     set_param([gcb '/fltIDcQReq'], 'Port', '4');
      |     set_param([gcb '/fltIAcReq'], 'Port', '5');
      |     set_param([gcb '/u16FAc'], 'Port', '6');
      |     set_param([gcb '/u8LdqSwitch'], 'Port', '7');
      | 
      | 
      |     if (posblk(4) - posblk(2)) < 200
      |       height = 200;
      |       set_param(gcb,'Position',[posblk(1), posblk(2), posblk(3), posblk(2)+height])
      |     end
      |   end
      | end
      | if (cfg == 1)
      |   if strcmp(get_param([gcb '/fltR'], 'BlockType'), 'Terminator') || strcmp(get_param([gcb '/pLdqTable'], 'BlockType'), 'Outport')
      |     if strcmp(get_param([gcb '/fltR'], 'BlockType'), 'Terminator')
      |       pos = get_param([gcb, '/fltR'], 'Position');
      |       orient = get_param([gcb, '/fltR'], 'Orientation');
      |       delete_block([gcb, '/fltR']);
      |       add_block('built-in/Outport', [gcb '/fltR'], 'Position', pos, 'Orientation', orient);
      |     end
      | 
      |     if strcmp(get_param([gcb '/fltUdt'], 'BlockType'), 'Terminator')
      |       pos = get_param([gcb, '/fltUdt'], 'Position');
      |       orient = get_param([gcb, '/fltUdt'], 'Orientation');
      |       delete_block([gcb, '/fltUdt']);
      |       add_block('built-in/Outport', [gcb '/fltUdt'], 'Position', pos, 'Orientation', orient);
      |     end
      | 
      |     if strcmp(get_param([gcb '/pLdqTable'], 'BlockType'), 'Outport')
      |       pos = get_param([gcb, '/pLdqTable'], 'Position');
      |       orient = get_param([gcb, '/pLdqTable'], 'Orientation');
      |       delete_block([gcb, '/pLdqTable']);
      |       add_block('built-in/Terminator', [gcb, '/pLdqTable'], 'Position', pos, 'Orientation', orient);
      |     end
      | 
      |     set_param([gcb '/returnStatus'], 'Port', '1');
      |     set_param([gcb '/pUAlBeReq'], 'Port', '2');
      |     set_param([gcb '/fltLd'], 'Port', '3');
      |     set_param([gcb '/fltLq'], 'Port', '4');
      |     set_param([gcb '/fltR'], 'Port', '5');
      |     set_param([gcb '/fltUdt'], 'Port', '6');
      |   end
      | end
      | if (cfg == 2) || (cfg == 3)
      |   if strcmp(get_param([gcb '/pLdqTable'], 'BlockType'), 'Terminator')
      |     if strcmp(get_param([gcb '/fltR'], 'BlockType'), 'Terminator')
      |       pos = get_param([gcb, '/fltR'], 'Position');
      |       orient = get_param([gcb, '/fltR'], 'Orientation');
      |       delete_block([gcb, '/fltR']);
      |       add_block('built-in/Outport', [gcb '/fltR'], 'Position', pos, 'Orientation', orient);
      |     end
      | 
      |     if strcmp(get_param([gcb '/fltUdt'], 'BlockType'), 'Terminator')
      |       pos = get_param([gcb, '/fltUdt'], 'Position');
      |       orient = get_param([gcb, '/fltUdt'], 'Orientation');
      |       delete_block([gcb, '/fltUdt']);
      |       add_block('built-in/Outport', [gcb '/fltUdt'], 'Position', pos, 'Orientation', orient);
      |     end
      | 
      |     if strcmp(get_param([gcb '/pLdqTable'], 'BlockType'), 'Terminator')
      |       pos = get_param([gcb, '/pLdqTable'], 'Position');
      |       orient = get_param([gcb, '/pLdqTable'], 'Orientation');
      |       delete_block([gcb, '/pLdqTable']);
      |       add_block('built-in/Outport', [gcb '/pLdqTable'], 'Position', pos, 'Orientation', orient);
      |     end
      | 
      |     set_param([gcb '/returnStatus'], 'Port', '1');
      |     set_param([gcb '/pUAlBeReq'], 'Port', '2');
      |     set_param([gcb '/fltLd'], 'Port', '3');
      |     set_param([gcb '/fltLq'], 'Port', '4');
      |     set_param([gcb '/fltR'], 'Port', '5');
      |     set_param([gcb '/fltUdt'], 'Port', '6');
      |     set_param([gcb '/pLdqTable'], 'Port', '7');
      |   end
      | end
      | if (cfg == 4)
      |   if strcmp(get_param([gcb '/fltR'], 'BlockType'), 'Outport')
      |     if strcmp(get_param([gcb '/fltR'], 'BlockType'), 'Outport')
      |       pos = get_param([gcb, '/fltR'], 'Position');
      |       orient = get_param([gcb, '/fltR'], 'Orientation');
      |       delete_block([gcb, '/fltR']);
      |       add_block('built-in/Terminator', [gcb, '/fltR'], 'Position', pos, 'Orientation', orient);
      |     end
      | 
      |     if strcmp(get_param([gcb '/fltUdt'], 'BlockType'), 'Outport')
      |       pos = get_param([gcb, '/fltUdt'], 'Position');
      |       orient = get_param([gcb, '/fltUdt'], 'Orientation');
      |       delete_block([gcb, '/fltUdt']);
      |       add_block('built-in/Terminator', [gcb, '/fltUdt'], 'Position', pos, 'Orientation', orient);
      |     end
      | 
      |     if strcmp(get_param([gcb '/pLdqTable'], 'BlockType'), 'Outport')
      |       pos = get_param([gcb, '/pLdqTable'], 'Position');
      |       orient = get_param([gcb, '/pLdqTable'], 'Orientation');
      |       delete_block([gcb, '/pLdqTable']);
      |       add_block('built-in/Terminator', [gcb, '/pLdqTable'], 'Position', pos, 'Orientation', orient);
      |     end
      | 
      |     set_param([gcb '/returnStatus'], 'Port', '1');
      |     set_param([gcb '/pUAlBeReq'], 'Port', '2');
      |     set_param([gcb '/fltLd'], 'Port', '3');
      |     set_param([gcb '/fltLq'], 'Port', '4');
      |   end
      | end
      settings: RTWSystemCode=Inline
      mask Help: web([fileparts(which('ammclib_bam_S32K3xx.slx')) '/../doc/S32K3XXMCLUG.pdf'], '-browser')
      mask TypeOptions cfg: DEFAULT | CFG1 | CFG2 | CFG3
      mask Callback cfg:
      | maskStr = get_param(gcb,'cfg');
      | if strcmp(maskStr,'DEFAULT')
      |   set_param(gcb,'MaskEnables',{'on','on','off','off','off','off','on'});
      | end
      | if strcmp(maskStr,'CFG1')
      |   set_param(gcb,'MaskEnables',{'on','on','on','off','on','off','on'});
      | end
      | if strcmp(maskStr,'CFG2')
      |   set_param(gcb,'MaskEnables',{'on','on','on','on','on','on','on'});
      | end
      | if strcmp(maskStr,'CFG3')
      |   set_param(gcb,'MaskEnables',{'on','off','off','off','off','off','on'});
      | end
      mask Display: pos = get_param(gcb, 'Position');width = pos(3) - pos(1); height = pos(4) - pos(2);tX=width/2;tY=height - 8;color('black');text(tX,tY, 'AMCLIB_EstimRL_FLT', 'horizontalAlignment', 'center');
  AMCLIB_FWSpeedLoop_FLT : Subsystem  StartFcn=|  TreatAsAtomicUnit=on  mask(AMCLIB_FWSpeedLoop_FLT){showStates=Hide (faster execution), resetStatesEnable=Pre-set according to the first set of inputs after reset, showDebugOutputs=Hide, fltState_Out_showOutput=off, SampleTime=-1, wf0=30, wksi=1, J=1.6e-5, Kt=0.067, lambdaW=0.9, lambdaFW=0.9, Idmax=-5, imax=10, udcbus=12, ramprpm=6, mechspeed=3000, polepairs=1, autoCalcEn=on, fltUmaxDivImax=0, fltLambdaW=0, fltLambdaFW=0, fltPropGainQ=0, fltIntegGainQ=0, fltLowerLimitQ=0, fltUpperLimitQ=0, fltPropGainFW=0, fltIntegGainFW=0, fltLowerLimitFW=0, fltUpperLimitFW=0, fltRampUp=0, fltRampDown=0, SampleTime_1=NaN}
      | ts=get_param(gcb,'CompiledSampleTime');
      | if iscell(ts)
      |   ts=ts{1};
      |   if iscell(ts)
      |     ts=ts{1};
      |   end
      | end
      | ts=ts(1);
      | set_param(gcb,'SampleTime_1',num2str(ts));
      | p=Simulink.Mask.get(gcb);
      | hintText=p.getDialogControl('timeHint');
      | SampleTime=Simulink.data.evalinGlobal(bdroot,get_param(gcb,'SampleTime'));
      | p=Simulink.Mask.get(gcb);
      | autoCalcEn=get_param(gcb,'autoCalcEn');
      | if strcmp(autoCalcEn,'on')
      |   if SampleTime==-1
      |     hintText.Prompt='Caution: Implementation parameters depend on inherited sample time. Make sure that the sample time of the block''s inputs corresponds to the sampling period in the target application.';
      |   else
      |     hintText.Prompt='Caution: Implementation parameters depend on the sample time. Make sure that the simulation time step corresponds to the sampling period in the target application.';
      |   end
      |   SampleTime=ts;
      |   fltUmaxDivImax_bkup=get_param(gcb,'fltUmaxDivImax');
      |   fltLambdaW_bkup=get_param(gcb,'fltLambdaW');
      |   fltLambdaFW_bkup=get_param(gcb,'fltLambdaFW');
      |   fltPropGainQ_bkup=get_param(gcb,'fltPropGainQ');
      |   fltIntegGainQ_bkup=get_param(gcb,'fltIntegGainQ');
      |   fltLowerLimitQ_bkup=get_param(gcb,'fltLowerLimitQ');
      |   fltUpperLimitQ_bkup=get_param(gcb,'fltUpperLimitQ');
      |   fltPropGainFW_bkup=get_param(gcb,'fltPropGainFW');
      |   fltIntegGainFW_bkup=get_param(gcb,'fltIntegGainFW');
      |   fltLowerLimitFW_bkup=get_param(gcb,'fltLowerLimitFW');
      |   fltUpperLimitFW_bkup=get_param(gcb,'fltUpperLimitFW');
      |   fltRampUp_bkup=get_param(gcb,'fltRampUp');
      |   fltRampDown_bkup=get_param(gcb,'fltRampDown');
      |   wf0=Simulink.data.evalinGlobal(bdroot,get_param(gcb,'wf0'));
      |   wksi=Simulink.data.evalinGlobal(bdroot,get_param(gcb,'wksi'));
      |   J=Simulink.data.evalinGlobal(bdroot,get_param(gcb,'J'));
      |   Kt=Simulink.data.evalinGlobal(bdroot,get_param(gcb,'Kt'));
      |   lambdaW=Simulink.data.evalinGlobal(bdroot,get_param(gcb,'lambdaW'));
      |   lambdaFW=Simulink.data.evalinGlobal(bdroot,get_param(gcb,'lambdaFW'));
      |   Idmax=Simulink.data.evalinGlobal(bdroot,get_param(gcb,'Idmax'));
      |   imax=Simulink.data.evalinGlobal(bdroot,get_param(gcb,'imax'));
      |   udcbus=Simulink.data.evalinGlobal(bdroot,get_param(gcb,'udcbus'));
      |   ramprpm=Simulink.data.evalinGlobal(bdroot,get_param(gcb,'ramprpm'));
      |   mechspeed=Simulink.data.evalinGlobal(bdroot,get_param(gcb,'mechspeed'));
      |   polepairs=Simulink.data.evalinGlobal(bdroot,get_param(gcb,'polepairs'));
      |   if (wf0<=0)
      |     warning('Natural frequency f0 must be positive.');
      |   end
      |   if (wksi<=0)
      |     warning('Current loop attenuation must be positive.');
      |   end
      |   if (wksi>1)
      |     warning('Current loop attenuation must not exceed 1.');
      |   end
      |   if (J<=0)
      |     warning('Moment of inertia J must be positive.');
      |   end
      |   if (Kt<=0)
      |     warning('Torque constant Kt must be positive.');
      |   end
      |   if (lambdaW<0)
      |     warning('MA filter smoothing factor must be in the range 0..1.');
      |   end
      |   if (lambdaW>1)
      |     warning('MA filter smoothing factor must be in the range 0..1.');
      |   end
      |   if (lambdaFW<0)
      |     warning('MA filter smoothing factor must be in the range 0..1.');
      |   end
      |   if (lambdaFW>1)
      |     warning('MA filter smoothing factor must be in the range 0..1.');
      |   end
      |   if (udcbus<=0)
      |     warning('DC bus voltage must be positive.');
      |   end
      |   if (imax<=0)
      |     warning('Max. phase current must be positive.');
      |   end
      |   if (mechspeed<=0)
      |     warning('Max. speed must be positive.');
      |   end
      |   if (polepairs<1)
      |     warning('Number of pole pairs must be a natural number (1, 2, 3, ...).');
      |   end
      |   if (round(polepairs)~=polepairs)
      |     warning('Number of pole pairs must be a natural number (1, 2, 3, ...).');
      |   end
      |   w0=6.283185307179586*wf0;
      |   pgain=2.0*wksi*w0*J/Kt;
      |   igain=w0*w0*J/Kt;
      |   wmax=polepairs*mechspeed*0.1047197551196598;
      |   fltPropGainQ=pgain;
      |   fltIntegGainQ=igain*SampleTime*0.5;
      |   fltLowerLimitQ=-wmax;
      |   fltUpperLimitQ=wmax;
      |   fltPropGainFW=0.9*pgain;
      |   fltIntegGainFW=fltIntegGainQ;
      |   if (Idmax<0)
      |     iratio=Idmax/imax;
      |     iratio=abs(iratio);
      |     if (abs(iratio) > 1)
      |       iratio = 0;
      |     end
      |     lowlim=acos(iratio)-1.570796326794897;
      |   else
      |     lowlim=0.0;
      |   end
      |   fltLowerLimitFW=lowlim;
      |   fltUpperLimitFW=0.0;
      |   fltLambdaW=lambdaW;
      |   fltLambdaFW=lambdaFW;
      |   rampsc=polepairs*abs(ramprpm)*0.1047197551196598;
      |   fltRampUp=rampsc;
      |   fltRampDown=rampsc;
      |   fltUmaxDivImax=0.5773502691896258*udcbus/imax;
      |   if isnan(fltUmaxDivImax)
      |     if ~strcmp(fltUmaxDivImax_bkup,'0')
      |       set_param(gcb,'fltUmaxDivImax','0');
      |     end
      |   else
      |     tmps=num2str(fltUmaxDivImax);
      |     if ~strcmp(fltUmaxDivImax_bkup,tmps)
      |       set_param(gcb,'fltUmaxDivImax',tmps);
      |     end
      |   end
      |   if isnan(fltLambdaW)
      |     if ~strcmp(fltLambdaW_bkup,'0')
      |       set_param(gcb,'fltLambdaW','0');
      |     end
      |   else
      |     tmps=num2str(fltLambdaW);
      |     if ~strcmp(fltLambdaW_bkup,tmps)
      |       set_param(gcb,'fltLambdaW',tmps);
      |     end
      |   end
      |   if isnan(fltLambdaFW)
      |     if ~strcmp(fltLambdaFW_bkup,'0')
      |       set_param(gcb,'fltLambdaFW','0');
      |     end
      |   else
      |     tmps=num2str(fltLambdaFW);
      |     if ~strcmp(fltLambdaFW_bkup,tmps)
      |       set_param(gcb,'fltLambdaFW',tmps);
      |     end
      |   end
      |   if isnan(fltPropGainQ)
      |     if ~strcmp(fltPropGainQ_bkup,'0')
      |       set_param(gcb,'fltPropGainQ','0');
      |     end
      |   else
      |     tmps=num2str(fltPropGainQ);
      |     if ~strcmp(fltPropGainQ_bkup,tmps)
      |       set_param(gcb,'fltPropGainQ',tmps);
      |     end
      |   end
      |   if isnan(fltIntegGainQ)
      |     if ~strcmp(fltIntegGainQ_bkup,'0')
      |       set_param(gcb,'fltIntegGainQ','0');
      |     end
      |   else
      |     tmps=num2str(fltIntegGainQ);
      |     if ~strcmp(fltIntegGainQ_bkup,tmps)
      |       set_param(gcb,'fltIntegGainQ',tmps);
      |     end
      |   end
      |   if isnan(fltLowerLimitQ)
      |     if ~strcmp(fltLowerLimitQ_bkup,'0')
      |       set_param(gcb,'fltLowerLimitQ','0');
      |     end
      |   else
      |     tmps=num2str(fltLowerLimitQ);
      |     if ~strcmp(fltLowerLimitQ_bkup,tmps)
      |       set_param(gcb,'fltLowerLimitQ',tmps);
      |     end
      |   end
      |   if isnan(fltUpperLimitQ)
      |     if ~strcmp(fltUpperLimitQ_bkup,'0')
      |       set_param(gcb,'fltUpperLimitQ','0');
      |     end
      |   else
      |     tmps=num2str(fltUpperLimitQ);
      |     if ~strcmp(fltUpperLimitQ_bkup,tmps)
      |       set_param(gcb,'fltUpperLimitQ',tmps);
      |     end
      |   end
      |   if isnan(fltPropGainFW)
      |     if ~strcmp(fltPropGainFW_bkup,'0')
      |       set_param(gcb,'fltPropGainFW','0');
      |     end
      |   else
      |     tmps=num2str(fltPropGainFW);
      |     if ~strcmp(fltPropGainFW_bkup,tmps)
      |       set_param(gcb,'fltPropGainFW',tmps);
      |     end
      |   end
      |   if isnan(fltIntegGainFW)
      |     if ~strcmp(fltIntegGainFW_bkup,'0')
      |       set_param(gcb,'fltIntegGainFW','0');
      |     end
      |   else
      |     tmps=num2str(fltIntegGainFW);
      |     if ~strcmp(fltIntegGainFW_bkup,tmps)
      |       set_param(gcb,'fltIntegGainFW',tmps);
      |     end
      |   end
      |   if isnan(fltLowerLimitFW)
      |     if ~strcmp(fltLowerLimitFW_bkup,'0')
      |       set_param(gcb,'fltLowerLimitFW','0');
      |     end
      |   else
      |     tmps=num2str(fltLowerLimitFW);
      |     if ~strcmp(fltLowerLimitFW_bkup,tmps)
      |       set_param(gcb,'fltLowerLimitFW',tmps);
      |     end
      |   end
      |   if isnan(fltUpperLimitFW)
      |     if ~strcmp(fltUpperLimitFW_bkup,'0')
      |       set_param(gcb,'fltUpperLimitFW','0');
      |     end
      |   else
      |     tmps=num2str(fltUpperLimitFW);
      |     if ~strcmp(fltUpperLimitFW_bkup,tmps)
      |       set_param(gcb,'fltUpperLimitFW',tmps);
      |     end
      |   end
      |   if isnan(fltRampUp)
      |     if ~strcmp(fltRampUp_bkup,'0')
      |       set_param(gcb,'fltRampUp','0');
      |     end
      |   else
      |     tmps=num2str(fltRampUp);
      |     if ~strcmp(fltRampUp_bkup,tmps)
      |       set_param(gcb,'fltRampUp',tmps);
      |     end
      |   end
      |   if isnan(fltRampDown)
      |     if ~strcmp(fltRampDown_bkup,'0')
      |       set_param(gcb,'fltRampDown','0');
      |     end
      |   else
      |     tmps=num2str(fltRampDown);
      |     if ~strcmp(fltRampDown_bkup,tmps)
      |       set_param(gcb,'fltRampDown',tmps);
      |     end
      |   end
      | end
      mask prompts: showStates "Show internal states:"; resetStatesEnable "Internal state after reset:"; showDebugOutputs "Show debugging outputs:"; fltState_Out_showOutput "Output speed ramp state (fltState_Out)"; SampleTime "Sample time (-1 for inherited):"; wf0 "Speed loop natural frequency f0 [Hz]:"; wksi "Speed loop attenuation ξ:"; J "Moment of inertia J [kg*m^2]:"; Kt "Motor torque constant Kt [N*m/A]:"; lambdaW "Speed MA filter smoothing factor λ (0..1):"; lambdaFW "Field weakening MA filter smoothing factor λ (0..1):"; Idmax "Maximum negative d-axis current (demagnetization current - CAUTION!) [A]:"; imax "Maximum phase current [A]:"; udcbus "DC bus voltage [V]:"; ramprpm "Speed ramp slope [ΔRPM per speed loop iteration]:"; mechspeed "Maximum mechanical speed of the motor [RPM]:"; polepairs "Number of pole pairs of the motor:"; autoCalcEn "Calculate implementation parameters from physical parameters"; fltUmaxDivImax "fltUmaxDivImax (Maximal coil voltage divided by the maximal coil current):"; fltLambdaW "fltLambdaW (velocity GDFLIB_FilterMA - smoothing factor):"; fltLambdaFW "fltLambdaFW (FW GDFLIB_FilterMA - smoothing factor):"; fltPropGainQ "fltPropGainQ (q-axis GFLIB_ControllerPIpAW - proportional gain):"; fltIntegGainQ "fltIntegGainQ (q-axis GFLIB_ControllerPIpAW - integral gain):"; fltLowerLimitQ "fltLowerLimitQ (q-axis GFLIB_ControllerPIpAW - lower limit):"; fltUpperLimitQ "fltUpperLimitQ (q-axis GFLIB_ControllerPIpAW - upper limit):"; fltPropGainFW "fltPropGainFW (FW GFLIB_ControllerPIpAW - proportional gain):"; fltIntegGainFW "fltIntegGainFW (FW GFLIB_ControllerPIpAW - integral gain):"; fltLowerLimitFW "fltLowerLimitFW (FW GFLIB_ControllerPIpAW - lower limit):"; fltUpperLimitFW "fltUpperLimitFW (FW GFLIB_ControllerPIpAW - upper limit):"; fltRampUp "fltRampUp (Ramp up increment coefficient):"; fltRampDown "fltRampDown (Ramp up decrement coefficient):"; SampleTime_1 "Discrete sample time:"
      mask help: Speed loop controller with Field Weakening capability for the PMSM field-oriented control algorithm in single precision floating-point implementation. This block supports re-initialization of the internal state during simulation. If the block is reset, the outputs of the MA filters, PI controllers, and the ramp will be aligned with the inputs fltFilterMAWOut_preset, fltFilterMAFWOut_preset, fltControllerPIpAWQOut_preset, fltControllerPIpAWFWOut_preset, and fltRampOut_preset. Refer to the AMMCLIB User's Guide for further details.
      mask init:
      | ddName = get_param(bdroot,'DataDictionary');
      | if length(ddName)==0
      |   set_param(bdroot,'DataDictionary','ammclib_types.sldd');
      | else
      |   dd = Simulink.data.dictionary.open(ddName);
      |   data = getSection(dd,'Design Data');
      |   if ~exist(data,'SWLIBS_2Syst_F16')
      |     addDataSource(dd,'ammclib_types.sldd');
      |     saveChanges(dd);
      |   end
      | end
      | outputsChanged = 0;
      | 
      | if showStates == 1
      |   % hidden state variables
      |   if strcmp(get_param([gcb '/fltUmaxDivImax'], 'BlockType'), 'Inport')
      |     posblk = get_param(gcb, 'Position');
      | 
      |     pos = get_param([gcb, '/fltUmaxDivImax'], 'Position');
      |     orient = get_param([gcb, '/fltUmaxDivImax'], 'Orientation');
      |     delete_block([gcb, '/fltUmaxDivImax']);
      |     add_block('built-in/Ground', [gcb, '/fltUmaxDivImax'], 'Position', pos, 'Orientation', orient);
      | 
      |     pos = get_param([gcb, '/fltLambdaW'], 'Position');
      |     orient = get_param([gcb, '/fltLambdaW'], 'Orientation');
      |     delete_block([gcb, '/fltLambdaW']);
      |     add_block('built-in/Ground', [gcb, '/fltLambdaW'], 'Position', pos, 'Orientation', orient);
      | 
      |     pos = get_param([gcb, '/fltLambdaFW'], 'Position');
      |     orient = get_param([gcb, '/fltLambdaFW'], 'Orientation');
      |     delete_block([gcb, '/fltLambdaFW']);
      |     add_block('built-in/Ground', [gcb, '/fltLambdaFW'], 'Position', pos, 'Orientation', orient);
      | 
      |     pos = get_param([gcb, '/fltPropGainQ'], 'Position');
      |     orient = get_param([gcb, '/fltPropGainQ'], 'Orientation');
      |     delete_block([gcb, '/fltPropGainQ']);
      |     add_block('built-in/Ground', [gcb, '/fltPropGainQ'], 'Position', pos, 'Orientation', orient);
      | 
      |     pos = get_param([gcb, '/fltIntegGainQ'], 'Position');
      |     orient = get_param([gcb, '/fltIntegGainQ'], 'Orientation');
      |     delete_block([gcb, '/fltIntegGainQ']);
      |     add_block('built-in/Ground', [gcb, '/fltIntegGainQ'], 'Position', pos, 'Orientation', orient);
      | 
      |     pos = get_param([gcb, '/fltLowerLimitQ'], 'Position');
      |     orient = get_param([gcb, '/fltLowerLimitQ'], 'Orientation');
      |     delete_block([gcb, '/fltLowerLimitQ']);
      |     add_block('built-in/Ground', [gcb, '/fltLowerLimitQ'], 'Position', pos, 'Orientation', orient);
      | 
      |     pos = get_param([gcb, '/fltUpperLimitQ'], 'Position');
      |     orient = get_param([gcb, '/fltUpperLimitQ'], 'Orientation');
      |     delete_block([gcb, '/fltUpperLimitQ']);
      |     add_block('built-in/Ground', [gcb, '/fltUpperLimitQ'], 'Position', pos, 'Orientation', orient);
      | 
      |     pos = get_param([gcb, '/fltPropGainFW'], 'Position');
      |     orient = get_param([gcb, '/fltPropGainFW'], 'Orientation');
      |     delete_block([gcb, '/fltPropGainFW']);
      |     add_block('built-in/Ground', [gcb, '/fltPropGainFW'], 'Position', pos, 'Orientation', orient);
      | 
      |     pos = get_param([gcb, '/fltIntegGainFW'], 'Position');
      |     orient = get_param([gcb, '/fltIntegGainFW'], 'Orientation');
      |     delete_block([gcb, '/fltIntegGainFW']);
      |     add_block('built-in/Ground', [gcb, '/fltIntegGainFW'], 'Position', pos, 'Orientation', orient);
      | 
      |     pos = get_param([gcb, '/fltLowerLimitFW'], 'Position');
      |     orient = get_param([gcb, '/fltLowerLimitFW'], 'Orientation');
      |     delete_block([gcb, '/fltLowerLimitFW']);
      |     add_block('built-in/Ground', [gcb, '/fltLowerLimitFW'], 'Position', pos, 'Orientation', orient);
      | 
      |     pos = get_param([gcb, '/fltUpperLimitFW'], 'Position');
      |     orient = get_param([gcb, '/fltUpperLimitFW'], 'Orientation');
      |     delete_block([gcb, '/fltUpperLimitFW']);
      |     add_block('built-in/Ground', [gcb, '/fltUpperLimitFW'], 'Position', pos, 'Orientation', orient);
      | 
      |     pos = get_param([gcb, '/fltRampUp'], 'Position');
      |     orient = get_param([gcb, '/fltRampUp'], 'Orientation');
      |     delete_block([gcb, '/fltRampUp']);
      |     add_block('built-in/Ground', [gcb, '/fltRampUp'], 'Position', pos, 'Orientation', orient);
      | 
      |     pos = get_param([gcb, '/fltRampDown'], 'Position');
      |     orient = get_param([gcb, '/fltRampDown'], 'Orientation');
      |     delete_block([gcb, '/fltRampDown']);
      |     add_block('built-in/Ground', [gcb, '/fltRampDown'], 'Position', pos, 'Orientation', orient);
      | 
      |     pos = get_param([gcb, '/fltIQReqK_1'], 'Position');
      |     orient = get_param([gcb, '/fltIQReqK_1'], 'Orientation');
      |     delete_block([gcb, '/fltIQReqK_1']);
      |     add_block('built-in/Ground', [gcb, '/fltIQReqK_1'], 'Position', pos, 'Orientation', orient);
      | 
      |     pos = get_param([gcb, '/fltAccW'], 'Position');
      |     orient = get_param([gcb, '/fltAccW'], 'Orientation');
      |     delete_block([gcb, '/fltAccW']);
      |     add_block('built-in/Ground', [gcb, '/fltAccW'], 'Position', pos, 'Orientation', orient);
      | 
      |     pos = get_param([gcb, '/fltAccFW'], 'Position');
      |     orient = get_param([gcb, '/fltAccFW'], 'Orientation');
      |     delete_block([gcb, '/fltAccFW']);
      |     add_block('built-in/Ground', [gcb, '/fltAccFW'], 'Position', pos, 'Orientation', orient);
      | 
      |     pos = get_param([gcb, '/fltIntegPartK_1Q'], 'Position');
      |     orient = get_param([gcb, '/fltIntegPartK_1Q'], 'Orientation');
      |     delete_block([gcb, '/fltIntegPartK_1Q']);
      |     add_block('built-in/Ground', [gcb, '/fltIntegPartK_1Q'], 'Position', pos, 'Orientation', orient);
      | 
      |     pos = get_param([gcb, '/fltInK_1Q'], 'Position');
      |     orient = get_param([gcb, '/fltInK_1Q'], 'Orientation');
      |     delete_block([gcb, '/fltInK_1Q']);
      |     add_block('built-in/Ground', [gcb, '/fltInK_1Q'], 'Position', pos, 'Orientation', orient);
      | 
      |     pos = get_param([gcb, '/fltIntegPartK_1FW'], 'Position');
      |     orient = get_param([gcb, '/fltIntegPartK_1FW'], 'Orientation');
      |     delete_block([gcb, '/fltIntegPartK_1FW']);
      |     add_block('built-in/Ground', [gcb, '/fltIntegPartK_1FW'], 'Position', pos, 'Orientation', orient);
      | 
      |     pos = get_param([gcb, '/fltInK_1FW'], 'Position');
      |     orient = get_param([gcb, '/fltInK_1FW'], 'Orientation');
      |     delete_block([gcb, '/fltInK_1FW']);
      |     add_block('built-in/Ground', [gcb, '/fltInK_1FW'], 'Position', pos, 'Orientation', orient);
      | 
      |     pos = get_param([gcb, '/fltState'], 'Position');
      |     orient = get_param([gcb, '/fltState'], 'Orientation');
      |     delete_block([gcb, '/fltState']);
      |     add_block('built-in/Ground', [gcb, '/fltState'], 'Position', pos, 'Orientation', orient);
      | 
      | 
      |     pmask=Simulink.Mask.get(gcb);
      |     pctrl=pmask.getParameter('SampleTime');
      |     pctrl.set('TypeOptions',{'fltVelocityReq/SampleTime','fltVelocityFbck/SampleTime','fltIQFbck/SampleTime','fltUQReq/SampleTime','fltUQLim/SampleTime','fltFilterMAWOut_preset/SampleTime','fltFilterMAFWOut_preset/SampleTime','fltControllerPIpAWQOut_preset/SampleTime','fltControllerPIpAWFWOut_preset/SampleTime','fltRampOut_preset/SampleTime'});
      | 
      |     pos = get_param([gcb '/fltAccW_Out'], 'Position');
      |     orient = get_param([gcb '/fltAccW_Out'], 'Orientation');
      |     delete_block([gcb '/fltAccW_Out']);
      |     add_block('built-in/Terminator', [gcb '/fltAccW_Out'], 'Position', pos, 'Orientation', orient);
      | 
      |     pos = get_param([gcb '/fltAccFW_Out'], 'Position');
      |     orient = get_param([gcb '/fltAccFW_Out'], 'Orientation');
      |     delete_block([gcb '/fltAccFW_Out']);
      |     add_block('built-in/Terminator', [gcb '/fltAccFW_Out'], 'Position', pos, 'Orientation', orient);
      | 
      |     pos = get_param([gcb '/fltIntegPartK_1Q_Out'], 'Position');
      |     orient = get_param([gcb '/fltIntegPartK_1Q_Out'], 'Orientation');
      |     delete_block([gcb '/fltIntegPartK_1Q_Out']);
      |     add_block('built-in/Terminator', [gcb '/fltIntegPartK_1Q_Out'], 'Position', pos, 'Orientation', orient);
      | 
      |     pos = get_param([gcb '/fltInK_1Q_Out'], 'Position');
      |     orient = get_param([gcb '/fltInK_1Q_Out'], 'Orientation');
      |     delete_block([gcb '/fltInK_1Q_Out']);
      |     add_block('built-in/Terminator', [gcb '/fltInK_1Q_Out'], 'Position', pos, 'Orientation', orient);
      | 
      |     pos = get_param([gcb '/fltIntegPartK_1FW_Out'], 'Position');
      |     orient = get_param([gcb '/fltIntegPartK_1FW_Out'], 'Orientation');
      |     delete_block([gcb '/fltIntegPartK_1FW_Out']);
      |     add_block('built-in/Terminator', [gcb '/fltIntegPartK_1FW_Out'], 'Position', pos, 'Orientation', orient);
      | 
      |     pos = get_param([gcb '/fltInK_1FW_Out'], 'Position');
      |     orient = get_param([gcb '/fltInK_1FW_Out'], 'Orientation');
      |     delete_block([gcb '/fltInK_1FW_Out']);
      |     add_block('built-in/Terminator', [gcb '/fltInK_1FW_Out'], 'Position', pos, 'Orientation', orient);
      | 
      |     if strcmp(get_param([gcb '/fltWReqFilt'], 'BlockType'), 'Outport')
      |       pos = get_param([gcb '/fltWReqFilt'], 'Position');
      |       orient = get_param([gcb '/fltWReqFilt'], 'Orientation');
      |       delete_block([gcb '/fltWReqFilt']);
      |       add_block('built-in/Terminator', [gcb '/fltWReqFilt'], 'Position', pos, 'Orientation', orient);
      | 
      |       pos = get_param([gcb '/fltWErr'], 'Position');
      |       orient = get_param([gcb '/fltWErr'], 'Orientation');
      |       delete_block([gcb '/fltWErr']);
      |       add_block('built-in/Terminator', [gcb '/fltWErr'], 'Position', pos, 'Orientation', orient);
      | 
      |       pos = get_param([gcb '/fltIDQReqAmp'], 'Position');
      |       orient = get_param([gcb '/fltIDQReqAmp'], 'Orientation');
      |       delete_block([gcb '/fltIDQReqAmp']);
      |       add_block('built-in/Terminator', [gcb '/fltIDQReqAmp'], 'Position', pos, 'Orientation', orient);
      | 
      |       pos = get_param([gcb '/fltWFbckFilt'], 'Position');
      |       orient = get_param([gcb '/fltWFbckFilt'], 'Orientation');
      |       delete_block([gcb '/fltWFbckFilt']);
      |       add_block('built-in/Terminator', [gcb '/fltWFbckFilt'], 'Position', pos, 'Orientation', orient);
      | 
      |       pos = get_param([gcb '/fltIQErrSign'], 'Position');
      |       orient = get_param([gcb '/fltIQErrSign'], 'Orientation');
      |       delete_block([gcb '/fltIQErrSign']);
      |       add_block('built-in/Terminator', [gcb '/fltIQErrSign'], 'Position', pos, 'Orientation', orient);
      | 
      |       pos = get_param([gcb '/fltFWErr'], 'Position');
      |       orient = get_param([gcb '/fltFWErr'], 'Orientation');
      |       delete_block([gcb '/fltFWErr']);
      |       add_block('built-in/Terminator', [gcb '/fltFWErr'], 'Position', pos, 'Orientation', orient);
      | 
      |       pos = get_param([gcb '/fltIQErr'], 'Position');
      |       orient = get_param([gcb '/fltIQErr'], 'Orientation');
      |       delete_block([gcb '/fltIQErr']);
      |       add_block('built-in/Terminator', [gcb '/fltIQErr'], 'Position', pos, 'Orientation', orient);
      | 
      |       pos = get_param([gcb '/fltUQErr'], 'Position');
      |       orient = get_param([gcb '/fltUQErr'], 'Orientation');
      |       delete_block([gcb '/fltUQErr']);
      |       add_block('built-in/Terminator', [gcb '/fltUQErr'], 'Position', pos, 'Orientation', orient);
      | 
      |       pos = get_param([gcb '/fltFWErrFilt'], 'Position');
      |       orient = get_param([gcb '/fltFWErrFilt'], 'Orientation');
      |       delete_block([gcb '/fltFWErrFilt']);
      |       add_block('built-in/Terminator', [gcb '/fltFWErrFilt'], 'Position', pos, 'Orientation', orient);
      | 
      |       pos = get_param([gcb '/fltFWAngle'], 'Position');
      |       orient = get_param([gcb '/fltFWAngle'], 'Orientation');
      |       delete_block([gcb '/fltFWAngle']);
      |       add_block('built-in/Terminator', [gcb '/fltFWAngle'], 'Position', pos, 'Orientation', orient);
      | 
      |       pos = get_param([gcb '/fltFWSin'], 'Position');
      |       orient = get_param([gcb '/fltFWSin'], 'Orientation');
      |       delete_block([gcb '/fltFWSin']);
      |       add_block('built-in/Terminator', [gcb '/fltFWSin'], 'Position', pos, 'Orientation', orient);
      | 
      |       pos = get_param([gcb '/fltFWCos'], 'Position');
      |       orient = get_param([gcb '/fltFWCos'], 'Orientation');
      |       delete_block([gcb '/fltFWCos']);
      |       add_block('built-in/Terminator', [gcb '/fltFWCos'], 'Position', pos, 'Orientation', orient);
      | 
      |     end
      | 
      |     set_param([gcb '/fltVelocityReq'], 'Port', '1');
      |     set_param([gcb '/fltVelocityFbck'], 'Port', '2');
      |     set_param([gcb '/fltIQFbck'], 'Port', '3');
      |     set_param([gcb '/fltUQReq'], 'Port', '4');
      |     set_param([gcb '/fltUQLim'], 'Port', '5');
      |     set_param([gcb '/fltFilterMAWOut_preset'], 'Port', '6');
      |     set_param([gcb '/fltFilterMAFWOut_preset'], 'Port', '7');
      |     set_param([gcb '/fltControllerPIpAWQOut_preset'], 'Port', '8');
      |     set_param([gcb '/fltControllerPIpAWFWOut_preset'], 'Port', '9');
      |     set_param([gcb '/fltRampOut_preset'], 'Port', '10');
      | 
      |     tmpOutCnt=0;
      |     tmpOutCnt=tmpOutCnt+1;
      |     set_param([gcb '/pIDQReq'], 'Port', num2str(tmpOutCnt));
      |     tmpOutCnt=tmpOutCnt+1;
      |     set_param([gcb '/u16LimitFlagQ'], 'Port', num2str(tmpOutCnt));
      |     tmpOutCnt=tmpOutCnt+1;
      |     set_param([gcb '/u16LimitFlagFW'], 'Port', num2str(tmpOutCnt));
      |     if strcmp(get_param([gcb '/fltState_Out'], 'BlockType'), 'Outport')
